simulink model "FeedBack_Linearization"  (R2021b)
(part 3 of 9)

M = ft_5({q1,q2,t10,t1020,t1033,t1034,t1039,t1060,t1066,t1079,t1080,t1090,t1094,t1095,t1097,t1105,t1107,t1116,t1117,t1119,t112,t1120,t1124,t1125,t1131,t1132,t1136,t1140,t1146,t1149,t1151,t1155,t1159,t1168,t1179,t1182,t1183,t1189,t119,t1194,t1197,t1198,t120,t1203,t1204,t121,t1213,t122,t1222,t1229,t1232,t1250,t1255,t1269,t1272,t1282,t1284,t1287,t129,t1292,t1293,t13,t130,t1300,t1307,t1312,t132,t1324,t1327,t1333,t1337,t1338,t1340,t1341,t1342,t1348,t1359,t136,t1364,t1365,t1366,t1368,t1375,t1383,t1394,t1396,t1398,t14,t1403,t1404,t1410,t1414,t1417,t1419,t1425,t1426,t143,t1432,t1446,t1465,t1475,t1486,t1495,t1496,t1498,t1499,t15,t1500,t1501,t1502,t1504,t1505,t1506,t1507,t1510,t1511,t1512,t1513,t1518,t1519,t1522,t1523,t1526,t1529,t153,t1530,t1534,t1535,t1536,t1537,t1542,t1546,t1548,t155,t1550,t1551,t1552,t1555,t1556,t156,t1560,t1561,t1565,t1568,t1569,t1575,t1584,t1589,t1593,t1595,t1598,t16,t1600,t1601,t1603,t1604,t1605,t1606,t1607,t1609,t1610,t1612,t1614,t1615,t1616,t1618,t1620,t1621,t1625,t1626,t1627,t1629,t1631,t1632,t1633,t1637,t164,t1645,t1648,t165,t1653,t1658,t1659,t1662,t1665,t1669,t167,t1671,t1678,t1682,t1685,t1686,t1687,t1689,t1690,t1691,t1695,t1696,t1697,t1699,t17,t170,t1700,t1701,t1702,t1703,t1704,t1707,t1708,t1709,t1710,t1711,t1713,t1715,t1719,t172,t1725,t1726,t1729,t173,t1730,t1731,t1736,t1738,t1741,t1743,t1744,t1749,t1750,t1752,t1753,t1754,t1757,t1758,t1760,t1761,t1762,t1763,t1766,t1767,t1768,t1769,t1771,t1772,t1773,t1776,t1777,t1780,t1782,t1783,t1784,t1785,t1786,t1789,t1790,t1794,t1795,t1797,t1798,t18,t180,t1802,t1803,t1804,t1805,t1806,t1807,t1808,t1809,t1810,t1811,t1812,t1813,t1814,t1815,t1816,t1817,t1818,t1819,t1820,t1821,t1822,t1823,t1824,t1825,t1826,t1827,t1828,t1829,t1831,t1832,t1833,t1835,t1836,t1837,t1839,t1840,t1843,t1844,t1845,t1846,t1847,t1848,t1851,t1852,t1853,t1854,t1855,t1856,t1857,t1858,t1862,t1863,t1867,t1868,t1869,t1870,t1871,t1873,t1874,t1875,t1876,t1877,t1878,t1879,t1883,t1884,t1885,t1888,t1889,t1890,t1892,t1893,t1894,t1895,t1896,t1897,t1900,t1901,t1902,t1903,t1904,t1905,t1906,t1907,t191,t1912,t1913,t1914,t1915,t1916,t1917,t1918,t1919,t1920,t1921,t1922,t1923,t1924,t1925,t1926,t1927,t1929,t1930,t1931,t1932,t1933,t1935,t1937,t1939,t1940,t1941,t1942,t1943,t1944,t1945,t1946,t1947,t1948,t1949,t1950,t1951,t1952,t1953,t1954,t1955,t1956,t1957,t1958,t1959,t1960,t1961,t1962,t1963,t1964,t1965,t1966,t1967,t1969,t1970,t1972,t1973,t1974,t1975,t1976,t1977,t1980,t1981,t1983,t1984,t1985,t1986,t1987,t1990,t1991,t1992,t1993,t1996,t1997,t1998,t1999,t2000,t2001,t2002,t2003,t2004,t2005,t2006,t2007,t2008,t2009,t2011,t2013,t2016,t2017,t2018,t2019,t2021,t2024,t2025,t2027,t2029,t203,t2031,t2032,t2033,t2035,t2036,t2039,t2041,t2043,t2045,t2047,t2048,t2049,t205,t2051,t2054,t2055,t2056,t2057,t2059,t2060,t2062,t2063,t2064,t2065,t2066,t2067,t2068,t2070,t2072,t2073,t2075,t2077,t2079,t2080,t2081,t2082,t2083,t2084,t2088,t2089,t2090,t2091,t2093,t2094,t2095,t2096,t2098,t210,t2101,t2102,t2104,t2106,t2107,t2109,t2111,t2112,t2113,t2114,t2115,t2117,t2118,t2120,t2121,t2122,t2124,t2126,t2128,t2129,t2131,t2132,t2133,t2134,t2135,t2136,t2137,t2139,t2141,t2142,t2145,t2146,t2148,t2149,t2150,t2151,t2152,t2153,t2154,t2156,t2158,t2161,t2162,t2164,t2166,t2168,t2169,t2170,t2172,t2174,t2175,t2176,t2178,t2179,t2182,t2183,t2184,t2187,t2188,t2189,t2190,t2191,t2193,t2194,t2195,t2197,t2201,t2202,t2203,t2204,t2205,t2206,t2208,t2210,t2211,t2212,t2214,t2215,t2216,t2218,t2221,t2222,t2223,t2225,t2226,t2228,t2229,t223,t2231,t2232,t2234,t2235,t2236,t2237,t2239,t2241,t2242,t2244,t2246,t2248,t2249,t225,t2253,t2254,t2255,t2256,t2258,t2259,t2260,t2261,t2262,t2263,t2264,t2266,t2267,t2268,t2269,t227,t2271,t2272,t2273,t2274,t2276,t2278,t228,t2280,t2284,t2287,t2288,t2289,t2295,t2296,t2300,t2301,t2305,t2306,t2309,t231,t2310,t2311,t2313,t2315,t2316,t2318,t2320,t2323,t2324,t2328,t2329,t2331,t2332,t2334,t2335,t2337,t2339,t2340,t2341,t2343,t2344,t2345,t2347,t2348,t2351,t2355,t2356,t2358,t236,t2363,t2364,t2366,t2370,t2371,t2376,t2377,t2378,t2379,t2380,t2383,t2394,t2397,t2401,t2403,t2406,t2409,t2410,t2411,t2413,t2416,t2418,t2419,t2421,t2425,t2427,t2430,t2431,t2434,t2435,t2436,t2439,t2440,t2441,t2442,t2443,t2444,t2445,t2446,t2447,t2450,t2451,t2454,t2456,t2459,t246,t2461,t2462,t2466,t2471,t2472,t2475,t2476,t2478,t2479,t2480,t2492,t2495,t2496,t2497,t2501,t2504,t2505,t2506,t2510,t2511,t2512,t2515,t252,t2522,t2523,t2524,t2527,t2530,t2531,t2536,t2537,t2538,t2542,t2546,t2549,t2550,t2551,t2552,t2554,t2555,t2558,t2559,t2563,t2565,t2566,t257,t2571,t2573,t2575,t273,t277,t300,t308,t31,t311,t312,t313,t314,t315,t32,t328,t33,t333,t342,t346,t36,t395,t396,t397,t451,t452,t455,t470,t485,t5,t500,t51,t515,t53,t533,t544,t55,t565,t57,t580,t6,t614,t639,t648,t654,t655,t66,t671,t673,t675,t679,t68,t7,t703,t710,t711,t717,t725,t726,t727,t748,t75,t765,t769,t770,t773,t788,t795,t8,t822,t826,t836,t854,t856,t865,t87,t873,t888,t889,t890,t896,t9,t902,t909,t910,t914,t929,t930,t933,t938,t942,t944,t969,t977,t979,t98,t980});
end
function M = ft_5(ct)
q1 = ct{1};
q2 = ct{2};
t10 = ct{3};
t1020 = ct{4};
t1033 = ct{5};
t1034 = ct{6};
t1039 = ct{7};
t1060 = ct{8};
t1066 = ct{9};
t1079 = ct{10};
t1080 = ct{11};
t1090 = ct{12};
t1094 = ct{13};
t1095 = ct{14};
t1097 = ct{15};
t1105 = ct{16};
t1107 = ct{17};
t1116 = ct{18};
t1117 = ct{19};
t1119 = ct{20};
t112 = ct{21};
t1120 = ct{22};
t1124 = ct{23};
t1125 = ct{24};
t1131 = ct{25};
t1132 = ct{26};
t1136 = ct{27};
t1140 = ct{28};
t1146 = ct{29};
t1149 = ct{30};
t1151 = ct{31};
t1155 = ct{32};
t1159 = ct{33};
t1168 = ct{34};
t1179 = ct{35};
t1182 = ct{36};
t1183 = ct{37};
t1189 = ct{38};
t119 = ct{39};
t1194 = ct{40};
t1197 = ct{41};
t1198 = ct{42};
t120 = ct{43};
t1203 = ct{44};
t1204 = ct{45};
t121 = ct{46};
t1213 = ct{47};
t122 = ct{48};
t1222 = ct{49};
t1229 = ct{50};
t1232 = ct{51};
t1250 = ct{52};
t1255 = ct{53};
t1269 = ct{54};
t1272 = ct{55};
t1282 = ct{56};
t1284 = ct{57};
t1287 = ct{58};
t129 = ct{59};
t1292 = ct{60};
t1293 = ct{61};
t13 = ct{62};
t130 = ct{63};
t1300 = ct{64};
t1307 = ct{65};
t1312 = ct{66};
t132 = ct{67};
t1324 = ct{68};
t1327 = ct{69};
t1333 = ct{70};
t1337 = ct{71};
t1338 = ct{72};
t1340 = ct{73};
t1341 = ct{74};
t1342 = ct{75};
t1348 = ct{76};
t1359 = ct{77};
t136 = ct{78};
t1364 = ct{79};
t1365 = ct{80};
t1366 = ct{81};
t1368 = ct{82};
t1375 = ct{83};
t1383 = ct{84};
t1394 = ct{85};
t1396 = ct{86};
t1398 = ct{87};
t14 = ct{88};
t1403 = ct{89};
t1404 = ct{90};
t1410 = ct{91};
t1414 = ct{92};
t1417 = ct{93};
t1419 = ct{94};
t1425 = ct{95};
t1426 = ct{96};
t143 = ct{97};
t1432 = ct{98};
t1446 = ct{99};
t1465 = ct{100};
t1475 = ct{101};
t1486 = ct{102};
t1495 = ct{103};
t1496 = ct{104};
t1498 = ct{105};
t1499 = ct{106};
t15 = ct{107};
t1500 = ct{108};
t1501 = ct{109};
t1502 = ct{110};
t1504 = ct{111};
t1505 = ct{112};
t1506 = ct{113};
t1507 = ct{114};
t1510 = ct{115};
t1511 = ct{116};
t1512 = ct{117};
t1513 = ct{118};
t1518 = ct{119};
t1519 = ct{120};
t1522 = ct{121};
t1523 = ct{122};
t1526 = ct{123};
t1529 = ct{124};
t153 = ct{125};
t1530 = ct{126};
t1534 = ct{127};
t1535 = ct{128};
t1536 = ct{129};
t1537 = ct{130};
t1542 = ct{131};
t1546 = ct{132};
t1548 = ct{133};
t155 = ct{134};
t1550 = ct{135};
t1551 = ct{136};
t1552 = ct{137};
t1555 = ct{138};
t1556 = ct{139};
t156 = ct{140};
t1560 = ct{141};
t1561 = ct{142};
t1565 = ct{143};
t1568 = ct{144};
t1569 = ct{145};
t1575 = ct{146};
t1584 = ct{147};
t1589 = ct{148};
t1593 = ct{149};
t1595 = ct{150};
t1598 = ct{151};
t16 = ct{152};
t1600 = ct{153};
t1601 = ct{154};
t1603 = ct{155};
t1604 = ct{156};
t1605 = ct{157};
t1606 = ct{158};
t1607 = ct{159};
t1609 = ct{160};
t1610 = ct{161};
t1612 = ct{162};
t1614 = ct{163};
t1615 = ct{164};
t1616 = ct{165};
t1618 = ct{166};
t1620 = ct{167};
t1621 = ct{168};
t1625 = ct{169};
t1626 = ct{170};
t1627 = ct{171};
t1629 = ct{172};
t1631 = ct{173};
t1632 = ct{174};
t1633 = ct{175};
t1637 = ct{176};
t164 = ct{177};
t1645 = ct{178};
t1648 = ct{179};
t165 = ct{180};
t1653 = ct{181};
t1658 = ct{182};
t1659 = ct{183};
t1662 = ct{184};
t1665 = ct{185};
t1669 = ct{186};
t167 = ct{187};
t1671 = ct{188};
t1678 = ct{189};
t1682 = ct{190};
t1685 = ct{191};
t1686 = ct{192};
t1687 = ct{193};
t1689 = ct{194};
t1690 = ct{195};
t1691 = ct{196};
t1695 = ct{197};
t1696 = ct{198};
t1697 = ct{199};
t1699 = ct{200};
t17 = ct{201};
t170 = ct{202};
t1700 = ct{203};
t1701 = ct{204};
t1702 = ct{205};
t1703 = ct{206};
t1704 = ct{207};
t1707 = ct{208};
t1708 = ct{209};
t1709 = ct{210};
t1710 = ct{211};
t1711 = ct{212};
t1713 = ct{213};
t1715 = ct{214};
t1719 = ct{215};
t172 = ct{216};
t1725 = ct{217};
t1726 = ct{218};
t1729 = ct{219};
t173 = ct{220};
t1730 = ct{221};
t1731 = ct{222};
t1736 = ct{223};
t1738 = ct{224};
t1741 = ct{225};
t1743 = ct{226};
t1744 = ct{227};
t1749 = ct{228};
t1750 = ct{229};
t1752 = ct{230};
t1753 = ct{231};
t1754 = ct{232};
t1757 = ct{233};
t1758 = ct{234};
t1760 = ct{235};
t1761 = ct{236};
t1762 = ct{237};
t1763 = ct{238};
t1766 = ct{239};
t1767 = ct{240};
t1768 = ct{241};
t1769 = ct{242};
t1771 = ct{243};
t1772 = ct{244};
t1773 = ct{245};
t1776 = ct{246};
t1777 = ct{247};
t1780 = ct{248};
t1782 = ct{249};
t1783 = ct{250};
t1784 = ct{251};
t1785 = ct{252};
t1786 = ct{253};
t1789 = ct{254};
t1790 = ct{255};
t1794 = ct{256};
t1795 = ct{257};
t1797 = ct{258};
t1798 = ct{259};
t18 = ct{260};
t180 = ct{261};
t1802 = ct{262};
t1803 = ct{263};
t1804 = ct{264};
t1805 = ct{265};
t1806 = ct{266};
t1807 = ct{267};
t1808 = ct{268};
t1809 = ct{269};
t1810 = ct{270};
t1811 = ct{271};
t1812 = ct{272};
t1813 = ct{273};
t1814 = ct{274};
t1815 = ct{275};
t1816 = ct{276};
t1817 = ct{277};
t1818 = ct{278};
t1819 = ct{279};
t1820 = ct{280};
t1821 = ct{281};
t1822 = ct{282};
t1823 = ct{283};
t1824 = ct{284};
t1825 = ct{285};
t1826 = ct{286};
t1827 = ct{287};
t1828 = ct{288};
t1829 = ct{289};
t1831 = ct{290};
t1832 = ct{291};
t1833 = ct{292};
t1835 = ct{293};
t1836 = ct{294};
t1837 = ct{295};
t1839 = ct{296};
t1840 = ct{297};
t1843 = ct{298};
t1844 = ct{299};
t1845 = ct{300};
t1846 = ct{301};
t1847 = ct{302};
t1848 = ct{303};
t1851 = ct{304};
t1852 = ct{305};
t1853 = ct{306};
t1854 = ct{307};
t1855 = ct{308};
t1856 = ct{309};
t1857 = ct{310};
t1858 = ct{311};
t1862 = ct{312};
t1863 = ct{313};
t1867 = ct{314};
t1868 = ct{315};
t1869 = ct{316};
t1870 = ct{317};
t1871 = ct{318};
t1873 = ct{319};
t1874 = ct{320};
t1875 = ct{321};
t1876 = ct{322};
t1877 = ct{323};
t1878 = ct{324};
t1879 = ct{325};
t1883 = ct{326};
t1884 = ct{327};
t1885 = ct{328};
t1888 = ct{329};
t1889 = ct{330};
t1890 = ct{331};
t1892 = ct{332};
t1893 = ct{333};
t1894 = ct{334};
t1895 = ct{335};
t1896 = ct{336};
t1897 = ct{337};
t1900 = ct{338};
t1901 = ct{339};
t1902 = ct{340};
t1903 = ct{341};
t1904 = ct{342};
t1905 = ct{343};
t1906 = ct{344};
t1907 = ct{345};
t191 = ct{346};
t1912 = ct{347};
t1913 = ct{348};
t1914 = ct{349};
t1915 = ct{350};
t1916 = ct{351};
t1917 = ct{352};
t1918 = ct{353};
t1919 = ct{354};
t1920 = ct{355};
t1921 = ct{356};
t1922 = ct{357};
t1923 = ct{358};
t1924 = ct{359};
t1925 = ct{360};
t1926 = ct{361};
t1927 = ct{362};
t1929 = ct{363};
t1930 = ct{364};
t1931 = ct{365};
t1932 = ct{366};
t1933 = ct{367};
t1935 = ct{368};
t1937 = ct{369};
t1939 = ct{370};
t1940 = ct{371};
t1941 = ct{372};
t1942 = ct{373};
t1943 = ct{374};
t1944 = ct{375};
t1945 = ct{376};
t1946 = ct{377};
t1947 = ct{378};
t1948 = ct{379};
t1949 = ct{380};
t1950 = ct{381};
t1951 = ct{382};
t1952 = ct{383};
t1953 = ct{384};
t1954 = ct{385};
t1955 = ct{386};
t1956 = ct{387};
t1957 = ct{388};
t1958 = ct{389};
t1959 = ct{390};
t1960 = ct{391};
t1961 = ct{392};
t1962 = ct{393};
t1963 = ct{394};
t1964 = ct{395};
t1965 = ct{396};
t1966 = ct{397};
t1967 = ct{398};
t1969 = ct{399};
t1970 = ct{400};
t1972 = ct{401};
t1973 = ct{402};
t1974 = ct{403};
t1975 = ct{404};
t1976 = ct{405};
t1977 = ct{406};
t1980 = ct{407};
t1981 = ct{408};
t1983 = ct{409};
t1984 = ct{410};
t1985 = ct{411};
t1986 = ct{412};
t1987 = ct{413};
t1990 = ct{414};
t1991 = ct{415};
t1992 = ct{416};
t1993 = ct{417};
t1996 = ct{418};
t1997 = ct{419};
t1998 = ct{420};
t1999 = ct{421};
t2000 = ct{422};
t2001 = ct{423};
t2002 = ct{424};
t2003 = ct{425};
t2004 = ct{426};
t2005 = ct{427};
t2006 = ct{428};
t2007 = ct{429};
t2008 = ct{430};
t2009 = ct{431};
t2011 = ct{432};
t2013 = ct{433};
t2016 = ct{434};
t2017 = ct{435};
t2018 = ct{436};
t2019 = ct{437};
t2021 = ct{438};
t2024 = ct{439};
t2025 = ct{440};
t2027 = ct{441};
t2029 = ct{442};
t203 = ct{443};
t2031 = ct{444};
t2032 = ct{445};
t2033 = ct{446};
t2035 = ct{447};
t2036 = ct{448};
t2039 = ct{449};
t2041 = ct{450};
t2043 = ct{451};
t2045 = ct{452};
t2047 = ct{453};
t2048 = ct{454};
t2049 = ct{455};
t205 = ct{456};
t2051 = ct{457};
t2054 = ct{458};
t2055 = ct{459};
t2056 = ct{460};
t2057 = ct{461};
t2059 = ct{462};
t2060 = ct{463};
t2062 = ct{464};
t2063 = ct{465};
t2064 = ct{466};
t2065 = ct{467};
t2066 = ct{468};
t2067 = ct{469};
t2068 = ct{470};
t2070 = ct{471};
t2072 = ct{472};
t2073 = ct{473};
t2075 = ct{474};
t2077 = ct{475};
t2079 = ct{476};
t2080 = ct{477};
t2081 = ct{478};
t2082 = ct{479};
t2083 = ct{480};
t2084 = ct{481};
t2088 = ct{482};
t2089 = ct{483};
t2090 = ct{484};
t2091 = ct{485};
t2093 = ct{486};
t2094 = ct{487};
t2095 = ct{488};
t2096 = ct{489};
t2098 = ct{490};
t210 = ct{491};
t2101 = ct{492};
t2102 = ct{493};
t2104 = ct{494};
t2106 = ct{495};
t2107 = ct{496};
t2109 = ct{497};
t2111 = ct{498};
t2112 = ct{499};
t2113 = ct{500};
t2114 = ct{501};
t2115 = ct{502};
t2117 = ct{503};
t2118 = ct{504};
t2120 = ct{505};
t2121 = ct{506};
t2122 = ct{507};
t2124 = ct{508};
t2126 = ct{509};
t2128 = ct{510};
t2129 = ct{511};
t2131 = ct{512};
t2132 = ct{513};
t2133 = ct{514};
t2134 = ct{515};
t2135 = ct{516};
t2136 = ct{517};
t2137 = ct{518};
t2139 = ct{519};
t2141 = ct{520};
t2142 = ct{521};
t2145 = ct{522};
t2146 = ct{523};
t2148 = ct{524};
t2149 = ct{525};
t2150 = ct{526};
t2151 = ct{527};
t2152 = ct{528};
t2153 = ct{529};
t2154 = ct{530};
t2156 = ct{531};
t2158 = ct{532};
t2161 = ct{533};
t2162 = ct{534};
t2164 = ct{535};
t2166 = ct{536};
t2168 = ct{537};
t2169 = ct{538};
t2170 = ct{539};
t2172 = ct{540};
t2174 = ct{541};
t2175 = ct{542};
t2176 = ct{543};
t2178 = ct{544};
t2179 = ct{545};
t2182 = ct{546};
t2183 = ct{547};
t2184 = ct{548};
t2187 = ct{549};
t2188 = ct{550};
t2189 = ct{551};
t2190 = ct{552};
t2191 = ct{553};
t2193 = ct{554};
t2194 = ct{555};
t2195 = ct{556};
t2197 = ct{557};
t2201 = ct{558};
t2202 = ct{559};
t2203 = ct{560};
t2204 = ct{561};
t2205 = ct{562};
t2206 = ct{563};
t2208 = ct{564};
t2210 = ct{565};
t2211 = ct{566};
t2212 = ct{567};
t2214 = ct{568};
t2215 = ct{569};
t2216 = ct{570};
t2218 = ct{571};
t2221 = ct{572};
t2222 = ct{573};
t2223 = ct{574};
t2225 = ct{575};
t2226 = ct{576};
t2228 = ct{577};
t2229 = ct{578};
t223 = ct{579};
t2231 = ct{580};
t2232 = ct{581};
t2234 = ct{582};
t2235 = ct{583};
t2236 = ct{584};
t2237 = ct{585};
t2239 = ct{586};
t2241 = ct{587};
t2242 = ct{588};
t2244 = ct{589};
t2246 = ct{590};
t2248 = ct{591};
t2249 = ct{592};
t225 = ct{593};
t2253 = ct{594};
t2254 = ct{595};
t2255 = ct{596};
t2256 = ct{597};
t2258 = ct{598};
t2259 = ct{599};
t2260 = ct{600};
t2261 = ct{601};
t2262 = ct{602};
t2263 = ct{603};
t2264 = ct{604};
t2266 = ct{605};
t2267 = ct{606};
t2268 = ct{607};
t2269 = ct{608};
t227 = ct{609};
t2271 = ct{610};
t2272 = ct{611};
t2273 = ct{612};
t2274 = ct{613};
t2276 = ct{614};
t2278 = ct{615};
t228 = ct{616};
t2280 = ct{617};
t2284 = ct{618};
t2287 = ct{619};
t2288 = ct{620};
t2289 = ct{621};
t2295 = ct{622};
t2296 = ct{623};
t2300 = ct{624};
t2301 = ct{625};
t2305 = ct{626};
t2306 = ct{627};
t2309 = ct{628};
t231 = ct{629};
t2310 = ct{630};
t2311 = ct{631};
t2313 = ct{632};
t2315 = ct{633};
t2316 = ct{634};
t2318 = ct{635};
t2320 = ct{636};
t2323 = ct{637};
t2324 = ct{638};
t2328 = ct{639};
t2329 = ct{640};
t2331 = ct{641};
t2332 = ct{642};
t2334 = ct{643};
t2335 = ct{644};
t2337 = ct{645};
t2339 = ct{646};
t2340 = ct{647};
t2341 = ct{648};
t2343 = ct{649};
t2344 = ct{650};
t2345 = ct{651};
t2347 = ct{652};
t2348 = ct{653};
t2351 = ct{654};
t2355 = ct{655};
t2356 = ct{656};
t2358 = ct{657};
t236 = ct{658};
t2363 = ct{659};
t2364 = ct{660};
t2366 = ct{661};
t2370 = ct{662};
t2371 = ct{663};
t2376 = ct{664};
t2377 = ct{665};
t2378 = ct{666};
t2379 = ct{667};
t2380 = ct{668};
t2383 = ct{669};
t2394 = ct{670};
t2397 = ct{671};
t2401 = ct{672};
t2403 = ct{673};
t2406 = ct{674};
t2409 = ct{675};
t2410 = ct{676};
t2411 = ct{677};
t2413 = ct{678};
t2416 = ct{679};
t2418 = ct{680};
t2419 = ct{681};
t2421 = ct{682};
t2425 = ct{683};
t2427 = ct{684};
t2430 = ct{685};
t2431 = ct{686};
t2434 = ct{687};
t2435 = ct{688};
t2436 = ct{689};
t2439 = ct{690};
t2440 = ct{691};
t2441 = ct{692};
t2442 = ct{693};
t2443 = ct{694};
t2444 = ct{695};
t2445 = ct{696};
t2446 = ct{697};
t2447 = ct{698};
t2450 = ct{699};
t2451 = ct{700};
t2454 = ct{701};
t2456 = ct{702};
t2459 = ct{703};
t246 = ct{704};
t2461 = ct{705};
t2462 = ct{706};
t2466 = ct{707};
t2471 = ct{708};
t2472 = ct{709};
t2475 = ct{710};
t2476 = ct{711};
t2478 = ct{712};
t2479 = ct{713};
t2480 = ct{714};
t2492 = ct{715};
t2495 = ct{716};
t2496 = ct{717};
t2497 = ct{718};
t2501 = ct{719};
t2504 = ct{720};
t2505 = ct{721};
t2506 = ct{722};
t2510 = ct{723};
t2511 = ct{724};
t2512 = ct{725};
t2515 = ct{726};
t252 = ct{727};
t2522 = ct{728};
t2523 = ct{729};
t2524 = ct{730};
t2527 = ct{731};
t2530 = ct{732};
t2531 = ct{733};
t2536 = ct{734};
t2537 = ct{735};
t2538 = ct{736};
t2542 = ct{737};
t2546 = ct{738};
t2549 = ct{739};
t2550 = ct{740};
t2551 = ct{741};
t2552 = ct{742};
t2554 = ct{743};
t2555 = ct{744};
t2558 = ct{745};
t2559 = ct{746};
t2563 = ct{747};
t2565 = ct{748};
t2566 = ct{749};
t257 = ct{750};
t2571 = ct{751};
t2573 = ct{752};
t2575 = ct{753};
t273 = ct{754};
t277 = ct{755};
t300 = ct{756};
t308 = ct{757};
t31 = ct{758};
t311 = ct{759};
t312 = ct{760};
t313 = ct{761};
t314 = ct{762};
t315 = ct{763};
t32 = ct{764};
t328 = ct{765};
t33 = ct{766};
t333 = ct{767};
t342 = ct{768};
t346 = ct{769};
t36 = ct{770};
t395 = ct{771};
t396 = ct{772};
t397 = ct{773};
t451 = ct{774};
t452 = ct{775};
t455 = ct{776};
t470 = ct{777};
t485 = ct{778};
t5 = ct{779};
t500 = ct{780};
t51 = ct{781};
t515 = ct{782};
t53 = ct{783};
t533 = ct{784};
t544 = ct{785};
t55 = ct{786};
t565 = ct{787};
t57 = ct{788};
t580 = ct{789};
t6 = ct{790};
t614 = ct{791};
t639 = ct{792};
t648 = ct{793};
t654 = ct{794};
t655 = ct{795};
t66 = ct{796};
t671 = ct{797};
t673 = ct{798};
t675 = ct{799};
t679 = ct{800};
t68 = ct{801};
t7 = ct{802};
t703 = ct{803};
t710 = ct{804};
t711 = ct{805};
t717 = ct{806};
t725 = ct{807};
t726 = ct{808};
t727 = ct{809};
t748 = ct{810};
t75 = ct{811};
t765 = ct{812};
t769 = ct{813};
t770 = ct{814};
t773 = ct{815};
t788 = ct{816};
t795 = ct{817};
t8 = ct{818};
t822 = ct{819};
t826 = ct{820};
t836 = ct{821};
t854 = ct{822};
t856 = ct{823};
t865 = ct{824};
t87 = ct{825};
t873 = ct{826};
t888 = ct{827};
t889 = ct{828};
t890 = ct{829};
t896 = ct{830};
t9 = ct{831};
t902 = ct{832};
t909 = ct{833};
t910 = ct{834};
t914 = ct{835};
t929 = ct{836};
t930 = ct{837};
t933 = ct{838};
t938 = ct{839};
t942 = ct{840};
t944 = ct{841};
t969 = ct{842};
t977 = ct{843};
t979 = ct{844};
t98 = ct{845};
t980 = ct{846};
t2577 = t2478.*(-t826+t856.*(t129+t13.*(t51-t155))+t836.*(t156-t236)).*(-1.0./2.0);
et77 = t1394.*4.000000000000028e-5+t1518+t1530+t1593+t1709+t565.*(t129+t13.*(t51-t155)).*5.0e-5;
et78 = t225.*(t136-t246).*2.81e-3+t452.*(t57-t165).*5.0e-5;
et79 = t856.*(t66-t210).*2.81e-3;
t2580 = t1967.*(et77+et78+et79).*(-1.0./2.0);
et80 = t1394.*4.000000000000028e-5+t1518+t1530+t1593+t1709+t565.*(t129+t13.*(t51-t155)).*5.0e-5;
et81 = t225.*(t136-t246).*2.81e-3+t452.*(t57-t165).*5.0e-5;
et82 = t856.*(t66-t210).*2.81e-3;
t2581 = (t1967.*(et80+et81+et82))./2.0;
et83 = t1537+t1575+t1704-t1710+t396.*(t167+t7.*(t55-t130)).*3.0e-5+t565.*(t129+t13.*(t51-t155)).*5.000000000000004e-4;
et84 = t225.*(t136-t246).*5.0e-5+t452.*(t57-t165).*5.000000000000004e-4;
et85 = t856.*(t66-t210).*5.0e-5;
t2582 = ((et83+et84+et85).*(-t826+t856.*(t129+t13.*(t51-t155))+t836.*(t156-t236)))./2.0;
et86 = t710.*4.000000000000028e-5-t1375+t1486+t1535+t1542+t671.*(t129+t13.*(t51-t155)).*3.0e-5;
et87 = t655.*(t485+t7.*(t53-t132)).*2.32e-3+t888.*(t273+t14.*(t51-t155)).*2.32e-3;
et88 = t614.*(t156-t236).*3.0e-5;
t2584 = t1986.*(et86+et87+et88).*(-1.0./2.0);
et89 = t710.*4.000000000000028e-5-t1375+t1486+t1535+t1542+t671.*(t129+t13.*(t51-t155)).*3.0e-5;
et90 = t655.*(t485+t7.*(t53-t132)).*2.32e-3+t888.*(t273+t14.*(t51-t155)).*2.32e-3;
et91 = t614.*(t156-t236).*3.0e-5;
t2586 = (t1986.*(et89+et90+et91))./2.0;
et92 = t710.*4.000000000000028e-5-t1375+t1486+t1535+t1542+t671.*(t129+t13.*(t51-t155)).*3.0e-5;
et93 = t655.*(t485+t7.*(t53-t132)).*2.32e-3+t888.*(t273+t14.*(t51-t155)).*2.32e-3;
et94 = t614.*(t156-t236).*3.0e-5;
t2590 = t1990.*(et92+et93+et94).*(-1.0./2.0);
t1712 = -t1708;
t1714 = -t1711;
t1722 = -t1719;
t1733 = -t1726;
t1740 = -t1730;
t1746 = -t1741;
t1859 = -t1855;
t1860 = -t1856;
t1861 = -t1857;
t1864 = -t1858;
t1865 = -t1862;
t1866 = -t1863;
t1880 = -t1877;
t1881 = -t1878;
t1882 = -t1879;
t1898 = -t1893;
t1899 = -t1896;
t1908 = -t1901;
t1909 = -t1903;
t1910 = -t1904;
t1911 = -t1906;
t1934 = -t1932;
t1936 = -t1933;
t1938 = -t1937;
t1978 = -t1974;
t1979 = -t1976;
t1982 = -t1980;
t2012 = t1750+t1753;
t2014 = t1761+t1762;
t2050 = t1348+t1614+t1631;
t2069 = t1871+t1876;
t2125 = t1519+t1786+t1790;
t2180 = -t2179;
t2250 = t2006.*t2016.*3.5432e-1;
t2265 = t2006.*t2027.*3.5432e-1;
t2281 = t2003.*t2065.*3.5432e-1;
t2283 = t2006.*t2067.*3.5432e-1;
t2286 = -t2284;
t2290 = t2009.*t2065.*3.5432e-1;
t2291 = t2006.*t2072.*3.5432e-1;
t2292 = t2006.*(t203-t679+t725.*2.324e-2+t865+t873+t1146+t14.*(t143-t164).*1.9738e-1).*(-3.5432e-1);
t2294 = t2006.*(t203-t679+t725.*2.324e-2+t865+t873+t1146+t14.*(t143-t164).*1.9738e-1).*3.5432e-1;
t2297 = -t2296;
t2298 = t2016.*t2067.*3.5432e-1;
t2302 = -t2300;
t2304 = -t2301;
t2314 = t2019.*t2065.*3.5432e-1;
t2321 = t2027.*t2067.*3.5432e-1;
t2325 = -t2324;
t2346 = t2006.*t2126.*3.5432e-1;
t2349 = t2003.*t2136.*3.5432e-1;
t2352 = t2057.*t2065.*3.5432e-1;
t2359 = t2016.*t2126.*3.5432e-1;
t2360 = t2009.*t2136.*3.5432e-1;
t2361 = t2067.*t2072.*3.5432e-1;
t2362 = t2067.*(t203-t679+t725.*2.324e-2+t865+t873+t1146+t14.*(t143-t164).*1.9738e-1).*(-3.5432e-1);
t2365 = t2065.*t2082.*3.5432e-1;
t2372 = (t1398.*t2287)./2.0;
t2373 = t2027.*t2126.*3.5432e-1;
t2374 = t2019.*t2136.*3.5432e-1;
t2382 = t2067.*t2126.*3.5432e-1;
t2385 = t2057.*t2136.*3.5432e-1;
t2387 = t2072.*t2126.*3.5432e-1;
t2389 = t2126.*(t203-t679+t725.*2.324e-2+t865+t873+t1146+t14.*(t143-t164).*1.9738e-1).*(-3.5432e-1);
t2390 = t2126.*(t203-t679+t725.*2.324e-2+t865+t873+t1146+t14.*(t143-t164).*1.9738e-1).*3.5432e-1;
t2391 = t2065.*t2136.*3.5432e-1;
t2392 = t2082.*t2136.*3.5432e-1;
t2395 = (t1826.*t2280)./2.0;
t2398 = t2287.*(t1333+t888.*(t156-t236)).*(-1.0./2.0);
t2399 = (t2287.*(t1333+t888.*(t156-t236)))./2.0;
t2404 = (t1884.*t2280)./2.0;
t2408 = t2287.*(t639+t648.*(t129+t13.*(t51-t155))+t673.*(t156-t236)).*(-1.0./2.0);
t2414 = t2287.*(-t726+t671.*(t129+t13.*(t51-t155))+t614.*(t156-t236)).*(-1.0./2.0);
t2415 = t2287.*(t1107+t565.*(t129+t13.*(t51-t155))+t452.*(t57-t165)).*(-1.0./2.0);
t2420 = t2280.*(t1189+t225.*(t136-t246)+t856.*(t66-t210)).*(-1.0./2.0);
t2422 = (t1929.*t2280)./2.0;
t2423 = (t2280.*(t1189+t225.*(t136-t246)+t856.*(t66-t210)))./2.0;
t2429 = (t1967.*t2280)./2.0;
t2432 = (t1966.*t2288)./2.0;
t2437 = (t1973.*t2288)./2.0;
t2448 = (t1986.*t2288)./2.0;
t2452 = t2288.*(t890+t655.*(t485+t7.*(t53-t132))+t888.*(t273+t14.*(t51-t155))).*(-1.0./2.0);
t2453 = (t1990.*t2288)./2.0;
t2460 = (t1398.*t2413)./2.0;
t2464 = (t1738.*t2406)./2.0;
t2467 = t2413.*(t639+t648.*(t129+t13.*(t51-t155))+t673.*(t156-t236)).*(-1.0./2.0);
t2468 = t2413.*(-t726+t671.*(t129+t13.*(t51-t155))+t614.*(t156-t236)).*(-1.0./2.0);
t2469 = t2413.*(t1107+t565.*(t129+t13.*(t51-t155))+t452.*(t57-t165)).*(-1.0./2.0);
t2473 = -t2471;
t2482 = t1426+t1446+t1522+t1534+t1536+t1598+t1600+t1700+t1713;
t2483 = t1768.*(t1499+t1711+t1726-t1924+t396.*(t515+t15.*(t57-t165)).*7.950000000000001e-3+t1359.*(t485+t7.*(t53-t132)).*7.950000000000001e-3).*(-1.0./2.0);
t2484 = t2413.*(-t826+t856.*(t129+t13.*(t51-t155))+t836.*(t156-t236)).*(-1.0./2.0);
t2485 = (t2413.*(-t826+t856.*(t129+t13.*(t51-t155))+t836.*(t156-t236)))./2.0;
t2486 = (t1973.*t2406)./2.0;
t2488 = (t1986.*t2406)./2.0;
t2490 = t2406.*(t890+t655.*(t485+t7.*(t53-t132))+t888.*(t273+t14.*(t51-t155))).*(-1.0./2.0);
t2491 = (t1990.*t2406)./2.0;
t2493 = (t1826.*t2462)./2.0;
t2498 = -t2497;
t2499 = (t1884.*t2462)./2.0;
t2507 = t2462.*(t1189+t225.*(t136-t246)+t856.*(t66-t210)).*(-1.0./2.0);
t2508 = (t1929.*t2462)./2.0;
t2513 = (t1738.*t2476)./2.0;
t2516 = -t2515;
t2517 = (t1738.*t2479)./2.0;
t2518 = ((t1752+t1383.*(t485+t7.*(t53-t132))).*(t1495+t1708+t1730-t1921+t396.*(t515+t15.*(t57-t165)).*2.2e-4+t1359.*(t485+t7.*(t53-t132)).*2.2e-4))./2.0;
et95 = (t1743+t1368.*(t485+t7.*(t53-t132))).*(t1499+t1711+t1726-t1924+t396.*(t515+t15.*(t57-t165)).*7.950000000000001e-3+t1359.*(t485+t7.*(t53-t132)).*7.950000000000001e-3);
et96 = 1.0./2.0;
t2520 = et95.*et96;
t2525 = -t2524;
et97 = t1120+t1060.*(t485+t7.*(t53-t132))+t888.*(t257+t15.*(t273+t14.*(t51-t155)));
et98 = (t1499+t1711+t1726-t1924+t396.*(t515+t15.*(t57-t165)).*7.950000000000001e-3+t1359.*(t485+t7.*(t53-t132)).*7.950000000000001e-3)./2.0;
t2528 = et97.*et98;
t2539 = t2032.*(t1499+t1711+t1726-t1924+t396.*(t515+t15.*(t57-t165)).*7.950000000000001e-3+t1359.*(t485+t7.*(t53-t132)).*7.950000000000001e-3).*(-1.0./2.0);
et99 = t1203+t14.*t1383.*(t129+t13.*(t51-t155))+t14.*t1359.*(t156-t236);
et100 = (t1495+t1708+t1730-t1921+t396.*(t515+t15.*(t57-t165)).*2.2e-4+t1359.*(t485+t7.*(t53-t132)).*2.2e-4)./2.0;
t2540 = et99.*et100;
t2541 = -t2538;
et101 = t1179-t1618+t1105.*(t485+t7.*(t53-t132));
et102 = (t1499+t1711+t1726-t1924+t396.*(t515+t15.*(t57-t165)).*7.950000000000001e-3+t1359.*(t485+t7.*(t53-t132)).*7.950000000000001e-3)./2.0;
t2544 = et101.*et102;
t2545 = t2035.*(t1499+t1711+t1726-t1924+t396.*(t515+t15.*(t57-t165)).*7.950000000000001e-3+t1359.*(t485+t7.*(t53-t132)).*7.950000000000001e-3).*(-1.0./2.0);
t2553 = -t2552;
t2556 = t2049.*(t1495+t1708+t1730-t1921+t396.*(t515+t15.*(t57-t165)).*2.2e-4+t1359.*(t485+t7.*(t53-t132)).*2.2e-4).*(-1.0./2.0);
t2557 = (t2049.*(t1495+t1708+t1730-t1921+t396.*(t515+t15.*(t57-t165)).*2.2e-4+t1359.*(t485+t7.*(t53-t132)).*2.2e-4))./2.0;
et103 = (-t1614+t1626+t452.*(t515+t15.*(t57-t165))).*(t1495+t1708+t1730-t1921+t396.*(t515+t15.*(t57-t165)).*2.2e-4+t1359.*(t485+t7.*(t53-t132)).*2.2e-4);
et104 = 1.0./2.0;
t2560 = et103.*et104;
t2561 = t2051.*(t1495+t1708+t1730-t1921+t396.*(t515+t15.*(t57-t165)).*2.2e-4+t1359.*(t485+t7.*(t53-t132)).*2.2e-4).*(-1.0./2.0);
t2562 = (t2051.*(t1495+t1708+t1730-t1921+t396.*(t515+t15.*(t57-t165)).*2.2e-4+t1359.*(t485+t7.*(t53-t132)).*2.2e-4))./2.0;
t2567 = -t2566;
t2568 = (t1966.*t2476)./2.0;
t2576 = (t1966.*t2479)./2.0;
t2579 = (t1973.*t2476)./2.0;
t2583 = -t2582;
t2585 = (t1973.*t2479)./2.0;
t2587 = t2084.*(t1495+t1708+t1730-t1921+t396.*(t515+t15.*(t57-t165)).*2.2e-4+t1359.*(t485+t7.*(t53-t132)).*2.2e-4).*(-1.0./2.0);
t2589 = t2088.*(t1507+t1719+t1741-t1923+t396.*(t515+t15.*(t57-t165)).*2.900000000000001e-4+t1359.*(t485+t7.*(t53-t132)).*2.900000000000001e-4).*(-1.0./2.0);
t2591 = t2476.*(t890+t655.*(t485+t7.*(t53-t132))+t888.*(t273+t14.*(t51-t155))).*(-1.0./2.0);
t2592 = (t2476.*(t890+t655.*(t485+t7.*(t53-t132))+t888.*(t273+t14.*(t51-t155))))./2.0;
t2593 = (t1990.*t2476)./2.0;
t2595 = (t1986.*t2479)./2.0;
t2597 = t2479.*(t890+t655.*(t485+t7.*(t53-t132))+t888.*(t273+t14.*(t51-t155))).*(-1.0./2.0);
t2598 = t2113.*(t1507+t1719+t1741-t1923+t396.*(t515+t15.*(t57-t165)).*2.900000000000001e-4+t1359.*(t485+t7.*(t53-t132)).*2.900000000000001e-4).*(-1.0./2.0);
t2599 = t2120.*(t1507+t1719+t1741-t1923+t396.*(t515+t15.*(t57-t165)).*2.900000000000001e-4+t1359.*(t485+t7.*(t53-t132)).*2.900000000000001e-4).*(-1.0./2.0);
t2600 = t2121.*(t1507+t1719+t1741-t1923+t396.*(t515+t15.*(t57-t165)).*2.900000000000001e-4+t1359.*(t485+t7.*(t53-t132)).*2.900000000000001e-4).*(-1.0./2.0);
t2601 = (t2120.*(t1507+t1719+t1741-t1923+t396.*(t515+t15.*(t57-t165)).*2.900000000000001e-4+t1359.*(t485+t7.*(t53-t132)).*2.900000000000001e-4))./2.0;
t2602 = (t2121.*(t1507+t1719+t1741-t1923+t396.*(t515+t15.*(t57-t165)).*2.900000000000001e-4+t1359.*(t485+t7.*(t53-t132)).*2.900000000000001e-4))./2.0;
et105 = t1780-t1790+t889.*(t8.*(t57-t165)+t15.*(t136-t246));
et106 = (t1507+t1719+t1741-t1923+t396.*(t515+t15.*(t57-t165)).*2.900000000000001e-4+t1359.*(t485+t7.*(t53-t132)).*2.900000000000001e-4)./2.0;
t2603 = et105.*et106;
t2604 = t1282+t1496+t1511+t1686+t1701+t1888+t1895+t1913+t1920;
t2605 = t1287+t1498+t1506+t1702+t1703+t1889+t1907+t1914+t1925;
t2606 = t1307+t1510+t1513+t1685+t1696+t1890+t1892+t1917+t1922;
t2607 = t1768.*(t1901+t1906+t1974-t1975+t1368.*(t485+t7.*(t53-t132)).*7.950000000000001e-3+t1383.*(t485+t7.*(t53-t132)).*2.2e-4).*(-1.0./2.0);
t2608 = (t1768.*(t1901+t1906+t1974-t1975+t1368.*(t485+t7.*(t53-t132)).*7.950000000000001e-3+t1383.*(t485+t7.*(t53-t132)).*2.2e-4))./2.0;
t2609 = t1984.*(t1893+t1904+t1980-t1981+t1368.*(t485+t7.*(t53-t132)).*2.900000000000001e-4+t1383.*(t485+t7.*(t53-t132)).*2.9e-4).*(-1.0./2.0);
t2613 = t1584+t1609+t1758+t1820+t1827+t1836+t1846+t1942+t1957;
t2614 = t1589+t1610+t1767+t1821+t1824+t1837+t1843+t1946+t1963;
t2615 = t1595+t1612+t1763+t1818+t1829+t1840+t1854+t1940+t1955;
t2616 = t1548+t1615+t1725+t1844+t1845+t1868+t1873+t1951+t1956;
t2617 = t1551+t1616+t1744+t1847+t1848+t1869+t1874+t1958+t1962;
t2618 = t1561+t1620+t1729+t1852+t1853+t1870+t1875+t1950+t1959;
et107 = t1120+t1060.*(t485+t7.*(t53-t132))+t888.*(t257+t15.*(t273+t14.*(t51-t155)));
et108 = (t1901+t1906+t1974-t1975+t1368.*(t485+t7.*(t53-t132)).*7.950000000000001e-3+t1383.*(t485+t7.*(t53-t132)).*2.2e-4)./2.0;
t2622 = et107.*et108;
t2624 = t2032.*(t1901+t1906+t1974-t1975+t1368.*(t485+t7.*(t53-t132)).*7.950000000000001e-3+t1383.*(t485+t7.*(t53-t132)).*2.2e-4).*(-1.0./2.0);
t2625 = (t2032.*(t1901+t1906+t1974-t1975+t1368.*(t485+t7.*(t53-t132)).*7.950000000000001e-3+t1383.*(t485+t7.*(t53-t132)).*2.2e-4))./2.0;
et109 = t1203+t14.*t1383.*(t129+t13.*(t51-t155))+t14.*t1359.*(t156-t236);
et110 = (t1896+t1903+t1976-t1977+t1368.*(t485+t7.*(t53-t132)).*2.2e-4+t1383.*(t485+t7.*(t53-t132)).*1.089e-2)./2.0;
t2626 = et109.*et110;
et111 = t1179-t1618+t1105.*(t485+t7.*(t53-t132));
et112 = (t1901+t1906+t1974-t1975+t1368.*(t485+t7.*(t53-t132)).*7.950000000000001e-3+t1383.*(t485+t7.*(t53-t132)).*2.2e-4)./2.0;
t2627 = et111.*et112;
t2629 = t2035.*(t1901+t1906+t1974-t1975+t1368.*(t485+t7.*(t53-t132)).*7.950000000000001e-3+t1383.*(t485+t7.*(t53-t132)).*2.2e-4).*(-1.0./2.0);
t2630 = (t2035.*(t1901+t1906+t1974-t1975+t1368.*(t485+t7.*(t53-t132)).*7.950000000000001e-3+t1383.*(t485+t7.*(t53-t132)).*2.2e-4))./2.0;
t2631 = t2049.*(t1896+t1903+t1976-t1977+t1368.*(t485+t7.*(t53-t132)).*2.2e-4+t1383.*(t485+t7.*(t53-t132)).*1.089e-2).*(-1.0./2.0);
et113 = (-t1614+t1626+t452.*(t515+t15.*(t57-t165))).*(t1896+t1903+t1976-t1977+t1368.*(t485+t7.*(t53-t132)).*2.2e-4+t1383.*(t485+t7.*(t53-t132)).*1.089e-2);
et114 = 1.0./2.0;
t2632 = et113.*et114;
t2634 = t2051.*(t1896+t1903+t1976-t1977+t1368.*(t485+t7.*(t53-t132)).*2.2e-4+t1383.*(t485+t7.*(t53-t132)).*1.089e-2).*(-1.0./2.0);
t2637 = t2084.*(t1896+t1903+t1976-t1977+t1368.*(t485+t7.*(t53-t132)).*2.2e-4+t1383.*(t485+t7.*(t53-t132)).*1.089e-2).*(-1.0./2.0);
t2638 = (t2084.*(t1896+t1903+t1976-t1977+t1368.*(t485+t7.*(t53-t132)).*2.2e-4+t1383.*(t485+t7.*(t53-t132)).*1.089e-2))./2.0;
et115 = -t1766+t396.*(t515+t15.*(t57-t165))+t1359.*(t485+t7.*(t53-t132));
et116 = (t1901+t1906+t1974-t1975+t1368.*(t485+t7.*(t53-t132)).*7.950000000000001e-3+t1383.*(t485+t7.*(t53-t132)).*2.2e-4)./2.0;
t2639 = et115.*et116;
t2641 = t2088.*(t1893+t1904+t1980-t1981+t1368.*(t485+t7.*(t53-t132)).*2.900000000000001e-4+t1383.*(t485+t7.*(t53-t132)).*2.9e-4).*(-1.0./2.0);
t2642 = (t2088.*(t1893+t1904+t1980-t1981+t1368.*(t485+t7.*(t53-t132)).*2.900000000000001e-4+t1383.*(t485+t7.*(t53-t132)).*2.9e-4))./2.0;
t2647 = t2113.*(t1893+t1904+t1980-t1981+t1368.*(t485+t7.*(t53-t132)).*2.900000000000001e-4+t1383.*(t485+t7.*(t53-t132)).*2.9e-4).*(-1.0./2.0);
t2648 = (t2113.*(t1893+t1904+t1980-t1981+t1368.*(t485+t7.*(t53-t132)).*2.900000000000001e-4+t1383.*(t485+t7.*(t53-t132)).*2.9e-4))./2.0;
t2649 = t2120.*(t1893+t1904+t1980-t1981+t1368.*(t485+t7.*(t53-t132)).*2.900000000000001e-4+t1383.*(t485+t7.*(t53-t132)).*2.9e-4).*(-1.0./2.0);
t2650 = t2121.*(t1893+t1904+t1980-t1981+t1368.*(t485+t7.*(t53-t132)).*2.900000000000001e-4+t1383.*(t485+t7.*(t53-t132)).*2.9e-4).*(-1.0./2.0);
et117 = t1560-t1637-t1754+t1857+t1879-t1927-t1943+t1060.*(t485+t7.*(t53-t132)).*7.950000000000001e-3;
et118 = t888.*(t257+t15.*(t273+t14.*(t51-t155))).*7.950000000000001e-3;
t2651 = t1768.*(et117+et118).*(-1.0./2.0);
et119 = t1780-t1790+t889.*(t8.*(t57-t165)+t15.*(t136-t246));
et120 = (t1893+t1904+t1980-t1981+t1368.*(t485+t7.*(t53-t132)).*2.900000000000001e-4+t1383.*(t485+t7.*(t53-t132)).*2.9e-4)./2.0;
t2652 = et119.*et120;
et121 = -t1595+t1607+t1828+t1851-t1940-t1955+t675.*(t8.*(t57-t165)+t15.*(t136-t246)).*2.900000000000001e-4+t14.*t1383.*(t129+t13.*(t51-t155)).*2.2e-4;
et122 = t14.*t1359.*(t156-t236).*2.2e-4;
t2654 = t1768.*(et121+et122).*(-1.0./2.0);
et123 = -t1595+t1607+t1828+t1851-t1940-t1955+t675.*(t8.*(t57-t165)+t15.*(t136-t246)).*2.900000000000001e-4+t14.*t1383.*(t129+t13.*(t51-t155)).*2.2e-4;
et124 = t14.*t1359.*(t156-t236).*2.2e-4;
t2656 = (t1768.*(et123+et124))./2.0;
et125 = t1984.*(t1550-t1633-t1760+t1856+t1878-t1931-t1948+t1060.*(t485+t7.*(t53-t132)).*2.900000000000001e-4+t888.*(t257+t15.*(t273+t14.*(t51-t155))).*2.900000000000001e-4);
et126 = -1.0./2.0;
t2672 = et125.*et126;
et127 = t1984.*(t1550-t1633-t1760+t1856+t1878-t1931-t1948+t1060.*(t485+t7.*(t53-t132)).*2.900000000000001e-4+t888.*(t257+t15.*(t273+t14.*(t51-t155))).*2.900000000000001e-4);
et128 = 1.0./2.0;
t2673 = et127.*et128;
et129 = -t1589+t1605+t1819+t1831-t1946-t1963+t675.*(t8.*(t57-t165)+t15.*(t136-t246)).*2.94e-3+t14.*t1383.*(t129+t13.*(t51-t155)).*2.9e-4;
et130 = t14.*t1359.*(t156-t236).*2.9e-4;
t2674 = t1984.*(et129+et130).*(-1.0./2.0);
et131 = t1752+t1383.*(t485+t7.*(t53-t132));
et132 = t1546-t1632-t1749+t1855+t1877-t1926-t1944+t1060.*(t485+t7.*(t53-t132)).*2.2e-4+t888.*(t257+t15.*(t273+t14.*(t51-t155))).*2.2e-4;
et133 = 1.0./2.0;
t2684 = et131.*et132.*et133;
et134 = t1560-t1637-t1754+t1857+t1879-t1927-t1943+t1060.*(t485+t7.*(t53-t132)).*7.950000000000001e-3;
et135 = t888.*(t257+t15.*(t273+t14.*(t51-t155))).*7.950000000000001e-3;
t2686 = ((et134+et135).*(t1743+t1368.*(t485+t7.*(t53-t132))))./2.0;
et136 = -t1584+t1604+t1823+t1839-t1942-t1957+t675.*(t8.*(t57-t165)+t15.*(t136-t246)).*2.9e-4+t14.*t1383.*(t129+t13.*(t51-t155)).*1.089e-2;
et137 = t14.*t1359.*(t156-t236).*1.089e-2;
t2688 = ((et136+et137).*(t1752+t1383.*(t485+t7.*(t53-t132))))./2.0;
et138 = -t1595+t1607+t1828+t1851-t1940-t1955+t675.*(t8.*(t57-t165)+t15.*(t136-t246)).*2.900000000000001e-4+t14.*t1383.*(t129+t13.*(t51-t155)).*2.2e-4;
et139 = t14.*t1359.*(t156-t236).*2.2e-4;
t2689 = ((et138+et139).*(t1743+t1368.*(t485+t7.*(t53-t132))))./2.0;
et140 = -t1595+t1607+t1828+t1851-t1940-t1955+t675.*(t8.*(t57-t165)+t15.*(t136-t246)).*2.900000000000001e-4+t14.*t1383.*(t129+t13.*(t51-t155)).*2.2e-4;
et141 = t14.*t1359.*(t156-t236).*2.2e-4;
t2692 = ((et140+et141).*(t1120+t1060.*(t485+t7.*(t53-t132))+t888.*(t257+t15.*(t273+t14.*(t51-t155)))))./2.0;
et142 = t1560-t1637-t1754+t1857+t1879-t1927-t1943+t1060.*(t485+t7.*(t53-t132)).*7.950000000000001e-3;
et143 = t888.*(t257+t15.*(t273+t14.*(t51-t155))).*7.950000000000001e-3;
t2698 = t2032.*(et142+et143).*(-1.0./2.0);
et144 = t1203+t14.*t1383.*(t129+t13.*(t51-t155))+t14.*t1359.*(t156-t236);
et145 = t1546-t1632-t1749+t1855+t1877-t1926-t1944+t1060.*(t485+t7.*(t53-t132)).*2.2e-4+t888.*(t257+t15.*(t273+t14.*(t51-t155))).*2.2e-4;
et146 = 1.0./2.0;
t2699 = et144.*et145.*et146;
et147 = t1560-t1637-t1754+t1857+t1879-t1927-t1943+t1060.*(t485+t7.*(t53-t132)).*7.950000000000001e-3;
et148 = t888.*(t257+t15.*(t273+t14.*(t51-t155))).*7.950000000000001e-3;
t2701 = ((et147+et148).*(t1179-t1618+t1105.*(t485+t7.*(t53-t132))))./2.0;
et149 = t1560-t1637-t1754+t1857+t1879-t1927-t1943+t1060.*(t485+t7.*(t53-t132)).*7.950000000000001e-3;
et150 = t888.*(t257+t15.*(t273+t14.*(t51-t155))).*7.950000000000001e-3;
t2702 = t2035.*(et149+et150).*(-1.0./2.0);
et151 = -t1595+t1607+t1828+t1851-t1940-t1955+t675.*(t8.*(t57-t165)+t15.*(t136-t246)).*2.900000000000001e-4+t14.*t1383.*(t129+t13.*(t51-t155)).*2.2e-4;
et152 = t14.*t1359.*(t156-t236).*2.2e-4;
t2703 = t2032.*(et151+et152).*(-1.0./2.0);
et153 = -t1595+t1607+t1828+t1851-t1940-t1955+t675.*(t8.*(t57-t165)+t15.*(t136-t246)).*2.900000000000001e-4+t14.*t1383.*(t129+t13.*(t51-t155)).*2.2e-4;
et154 = t14.*t1359.*(t156-t236).*2.2e-4;
t2704 = (t2032.*(et153+et154))./2.0;
et155 = -t1595+t1607+t1828+t1851-t1940-t1955+t675.*(t8.*(t57-t165)+t15.*(t136-t246)).*2.900000000000001e-4+t14.*t1383.*(t129+t13.*(t51-t155)).*2.2e-4;
et156 = t14.*t1359.*(t156-t236).*2.2e-4;
t2705 = t2035.*(et155+et156).*(-1.0./2.0);
et157 = -t1595+t1607+t1828+t1851-t1940-t1955+t675.*(t8.*(t57-t165)+t15.*(t136-t246)).*2.900000000000001e-4+t14.*t1383.*(t129+t13.*(t51-t155)).*2.2e-4;
et158 = t14.*t1359.*(t156-t236).*2.2e-4;
t2706 = (t2035.*(et157+et158))./2.0;
et159 = t2049.*(t1546-t1632-t1749+t1855+t1877-t1926-t1944+t1060.*(t485+t7.*(t53-t132)).*2.2e-4+t888.*(t257+t15.*(t273+t14.*(t51-t155))).*2.2e-4);
et160 = -1.0./2.0;
t2709 = et159.*et160;
et161 = t2049.*(t1546-t1632-t1749+t1855+t1877-t1926-t1944+t1060.*(t485+t7.*(t53-t132)).*2.2e-4+t888.*(t257+t15.*(t273+t14.*(t51-t155))).*2.2e-4);
et162 = 1.0./2.0;
t2710 = et161.*et162;
et163 = -t1614+t1626+t452.*(t515+t15.*(t57-t165));
et164 = t1546-t1632-t1749+t1855+t1877-t1926-t1944+t1060.*(t485+t7.*(t53-t132)).*2.2e-4+t888.*(t257+t15.*(t273+t14.*(t51-t155))).*2.2e-4;
et165 = 1.0./2.0;
t2711 = et163.*et164.*et165;
et166 = -t1584+t1604+t1823+t1839-t1942-t1957+t675.*(t8.*(t57-t165)+t15.*(t136-t246)).*2.9e-4+t14.*t1383.*(t129+t13.*(t51-t155)).*1.089e-2;
et167 = t14.*t1359.*(t156-t236).*1.089e-2;
t2713 = t2049.*(et166+et167).*(-1.0./2.0);
et168 = -t1584+t1604+t1823+t1839-t1942-t1957+t675.*(t8.*(t57-t165)+t15.*(t136-t246)).*2.9e-4+t14.*t1383.*(t129+t13.*(t51-t155)).*1.089e-2;
et169 = t14.*t1359.*(t156-t236).*1.089e-2;
t2719 = ((et168+et169).*(-t1614+t1626+t452.*(t515+t15.*(t57-t165))))./2.0;
et170 = -t1584+t1604+t1823+t1839-t1942-t1957+t675.*(t8.*(t57-t165)+t15.*(t136-t246)).*2.9e-4+t14.*t1383.*(t129+t13.*(t51-t155)).*1.089e-2;
et171 = t14.*t1359.*(t156-t236).*1.089e-2;
t2720 = t2051.*(et170+et171).*(-1.0./2.0);
et172 = t2084.*(t1546-t1632-t1749+t1855+t1877-t1926-t1944+t1060.*(t485+t7.*(t53-t132)).*2.2e-4+t888.*(t257+t15.*(t273+t14.*(t51-t155))).*2.2e-4);
et173 = -1.0./2.0;
t2735 = et172.*et173;
et174 = t1560-t1637-t1754+t1857+t1879-t1927-t1943+t1060.*(t485+t7.*(t53-t132)).*7.950000000000001e-3;
et175 = t888.*(t257+t15.*(t273+t14.*(t51-t155))).*7.950000000000001e-3;
t2737 = ((et174+et175).*(-t1766+t396.*(t515+t15.*(t57-t165))+t1359.*(t485+t7.*(t53-t132))))./2.0;
et176 = -t1584+t1604+t1823+t1839-t1942-t1957+t675.*(t8.*(t57-t165)+t15.*(t136-t246)).*2.9e-4+t14.*t1383.*(t129+t13.*(t51-t155)).*1.089e-2;
et177 = t14.*t1359.*(t156-t236).*1.089e-2;
t2738 = t2084.*(et176+et177).*(-1.0./2.0);
et178 = -t1584+t1604+t1823+t1839-t1942-t1957+t675.*(t8.*(t57-t165)+t15.*(t136-t246)).*2.9e-4+t14.*t1383.*(t129+t13.*(t51-t155)).*1.089e-2;
et179 = t14.*t1359.*(t156-t236).*1.089e-2;
t2739 = (t2084.*(et178+et179))./2.0;
et180 = t2088.*(t1550-t1633-t1760+t1856+t1878-t1931-t1948+t1060.*(t485+t7.*(t53-t132)).*2.900000000000001e-4+t888.*(t257+t15.*(t273+t14.*(t51-t155))).*2.900000000000001e-4);
et181 = -1.0./2.0;
t2740 = et180.*et181;
et182 = -t1595+t1607+t1828+t1851-t1940-t1955+t675.*(t8.*(t57-t165)+t15.*(t136-t246)).*2.900000000000001e-4+t14.*t1383.*(t129+t13.*(t51-t155)).*2.2e-4;
et183 = t14.*t1359.*(t156-t236).*2.2e-4;
t2741 = ((et182+et183).*(-t1766+t396.*(t515+t15.*(t57-t165))+t1359.*(t485+t7.*(t53-t132))))./2.0;
et184 = -t1589+t1605+t1819+t1831-t1946-t1963+t675.*(t8.*(t57-t165)+t15.*(t136-t246)).*2.94e-3+t14.*t1383.*(t129+t13.*(t51-t155)).*2.9e-4;
et185 = t14.*t1359.*(t156-t236).*2.9e-4;
t2744 = t2088.*(et184+et185).*(-1.0./2.0);
et186 = -t1589+t1605+t1819+t1831-t1946-t1963+t675.*(t8.*(t57-t165)+t15.*(t136-t246)).*2.94e-3+t14.*t1383.*(t129+t13.*(t51-t155)).*2.9e-4;
et187 = t14.*t1359.*(t156-t236).*2.9e-4;
t2746 = (t2088.*(et186+et187))./2.0;
et188 = -t1589+t1605+t1819+t1831-t1946-t1963+t675.*(t8.*(t57-t165)+t15.*(t136-t246)).*2.94e-3+t14.*t1383.*(t129+t13.*(t51-t155)).*2.9e-4;
et189 = t14.*t1359.*(t156-t236).*2.9e-4;
t2757 = t2113.*(et188+et189).*(-1.0./2.0);
et190 = -t1589+t1605+t1819+t1831-t1946-t1963+t675.*(t8.*(t57-t165)+t15.*(t136-t246)).*2.94e-3+t14.*t1383.*(t129+t13.*(t51-t155)).*2.9e-4;
et191 = t14.*t1359.*(t156-t236).*2.9e-4;
t2758 = (t2113.*(et190+et191))./2.0;
et192 = t2120.*(t1550-t1633-t1760+t1856+t1878-t1931-t1948+t1060.*(t485+t7.*(t53-t132)).*2.900000000000001e-4+t888.*(t257+t15.*(t273+t14.*(t51-t155))).*2.900000000000001e-4);
et193 = -1.0./2.0;
t2759 = et192.*et193;
et194 = t2121.*(t1550-t1633-t1760+t1856+t1878-t1931-t1948+t1060.*(t485+t7.*(t53-t132)).*2.900000000000001e-4+t888.*(t257+t15.*(t273+t14.*(t51-t155))).*2.900000000000001e-4);
et195 = -1.0./2.0;
t2760 = et194.*et195;
et196 = t2120.*(t1550-t1633-t1760+t1856+t1878-t1931-t1948+t1060.*(t485+t7.*(t53-t132)).*2.900000000000001e-4+t888.*(t257+t15.*(t273+t14.*(t51-t155))).*2.900000000000001e-4);
et197 = 1.0./2.0;
t2761 = et196.*et197;
et198 = t2121.*(t1550-t1633-t1760+t1856+t1878-t1931-t1948+t1060.*(t485+t7.*(t53-t132)).*2.900000000000001e-4+t888.*(t257+t15.*(t273+t14.*(t51-t155))).*2.900000000000001e-4);
et199 = 1.0./2.0;
t2762 = et198.*et199;
et200 = -t1589+t1605+t1819+t1831-t1946-t1963+t675.*(t8.*(t57-t165)+t15.*(t136-t246)).*2.94e-3+t14.*t1383.*(t129+t13.*(t51-t155)).*2.9e-4;
et201 = t14.*t1359.*(t156-t236).*2.9e-4;
t2763 = t2121.*(et200+et201).*(-1.0./2.0);
et202 = t1780-t1790+t889.*(t8.*(t57-t165)+t15.*(t136-t246));
et203 = t1550-t1633-t1760+t1856+t1878-t1931-t1948+t1060.*(t485+t7.*(t53-t132)).*2.900000000000001e-4+t888.*(t257+t15.*(t273+t14.*(t51-t155))).*2.900000000000001e-4;
et204 = 1.0./2.0;
t2764 = et202.*et203.*et204;
et205 = -t1589+t1605+t1819+t1831-t1946-t1963+t675.*(t8.*(t57-t165)+t15.*(t136-t246)).*2.94e-3+t14.*t1383.*(t129+t13.*(t51-t155)).*2.9e-4;
et206 = t14.*t1359.*(t156-t236).*2.9e-4;
t2767 = ((et205+et206).*(t1780-t1790+t889.*(t8.*(t57-t165)+t15.*(t136-t246))))./2.0;
t2285 = -t2283;
t2293 = -t2291;
t2299 = -t2298;
t2322 = -t2321;
t2354 = -t2352;
t2367 = -t2365;
t2384 = -t2382;
t2386 = -t2385;
t2388 = -t2387;
t2393 = -t2392;
t2405 = -t2404;
t2438 = -t2437;
t2449 = -t2448;
t2455 = t1500+t1678+t1712+t1740+t1897+t1921;
t2457 = t1502+t1689+t1714+t1733+t1902+t1924;
t2458 = t1512+t1682+t1722+t1746+t1894+t1923;
t2487 = -t2486;
t2489 = -t2488;
t2494 = -t2493;
t2509 = -t2508;
t2514 = -t2513;
t2519 = -t2518;
t2521 = -t2520;
t2532 = t1899+t1905+t1909+t1915+t1977+t1979;
t2533 = t1908+t1911+t1912+t1918+t1975+t1978;
t2534 = t1898+t1900+t1910+t1916+t1981+t1982;
t2543 = -t2540;
t2569 = -t2568;
t2578 = t2069.*(t1507+t1719+t1741-t1923+t396.*(t515+t15.*(t57-t165)).*2.900000000000001e-4+t1359.*(t485+t7.*(t53-t132)).*2.900000000000001e-4).*(-1.0./2.0);
t2588 = -t2585;
t2594 = -t2593;
t2596 = -t2595;
t2610 = t1555+t1632+t1749+t1806+t1817+t1859+t1880+t1926+t1944;
t2611 = t1565+t1637+t1754+t1809+t1825+t1861+t1882+t1927+t1943;
t2612 = t1556+t1633+t1760+t1807+t1816+t1860+t1881+t1931+t1948;
t2619 = t1659+t1690+t1795+t1811+t1813+t1832+t1865+t1936+t1939;
t2620 = t1669+t1695+t1794+t1814+t1822+t1835+t1864+t1934+t1941;
t2621 = t1653+t1691+t1798+t1812+t1815+t1833+t1866+t1938+t1947;
t2623 = -t2622;
t2628 = -t2627;
t2633 = -t2632;
t2635 = (t1984.*t2605)./2.0;
t2640 = -t2639;
t2643 = t2604.*(t1752+t1383.*(t485+t7.*(t53-t132))).*(-1.0./2.0);
t2644 = (t2604.*(t1752+t1383.*(t485+t7.*(t53-t132))))./2.0;
t2645 = t2606.*(t1743+t1368.*(t485+t7.*(t53-t132))).*(-1.0./2.0);
t2646 = (t2606.*(t1743+t1368.*(t485+t7.*(t53-t132))))./2.0;
t2653 = t2606.*(t1120+t1060.*(t485+t7.*(t53-t132))+t888.*(t257+t15.*(t273+t14.*(t51-t155)))).*(-1.0./2.0);
t2655 = -t2652;
t2657 = (t2032.*t2606)./2.0;
t2658 = t2604.*(t1203+t14.*t1383.*(t129+t13.*(t51-t155))+t14.*t1359.*(t156-t236)).*(-1.0./2.0);
t2659 = (t2604.*(t1203+t14.*t1383.*(t129+t13.*(t51-t155))+t14.*t1359.*(t156-t236)))./2.0;
t2660 = t2606.*(t1179-t1618+t1105.*(t485+t7.*(t53-t132))).*(-1.0./2.0);
t2661 = (t2035.*t2606)./2.0;
t2662 = (t1768.*t2618)./2.0;
t2665 = (t2049.*t2604)./2.0;
t2667 = t2604.*(-t1614+t1626+t452.*(t515+t15.*(t57-t165))).*(-1.0./2.0);
t2668 = (t2051.*t2604)./2.0;
t2670 = (t2069.*t2605)./2.0;
t2671 = t2606.*(-t1766+t396.*(t515+t15.*(t57-t165))+t1359.*(t485+t7.*(t53-t132))).*(-1.0./2.0);
t2675 = (t2113.*t2605)./2.0;
t2676 = (t2120.*t2605)./2.0;
t2678 = (t2121.*t2605)./2.0;
t2679 = (t1984.*t2617)./2.0;
t2681 = t2605.*(t1780-t1790+t889.*(t8.*(t57-t165)+t15.*(t136-t246))).*(-1.0./2.0);
t2685 = -t2684;
t2687 = -t2686;
t2690 = t2616.*(t1752+t1383.*(t485+t7.*(t53-t132))).*(-1.0./2.0);
t2691 = t2618.*(t1743+t1368.*(t485+t7.*(t53-t132))).*(-1.0./2.0);
t2693 = -t2692;
t2700 = -t2699;
t2707 = t2618.*(t1120+t1060.*(t485+t7.*(t53-t132))+t888.*(t257+t15.*(t273+t14.*(t51-t155)))).*(-1.0./2.0);
t2708 = (t2618.*(t1120+t1060.*(t485+t7.*(t53-t132))+t888.*(t257+t15.*(t273+t14.*(t51-t155)))))./2.0;
t2714 = t2616.*(t1203+t14.*t1383.*(t129+t13.*(t51-t155))+t14.*t1359.*(t156-t236)).*(-1.0./2.0);
t2715 = t2618.*(t1179-t1618+t1105.*(t485+t7.*(t53-t132))).*(-1.0./2.0);
t2716 = (t2618.*(t1179-t1618+t1105.*(t485+t7.*(t53-t132))))./2.0;
t2717 = (t2035.*t2618)./2.0;
t2721 = -t2719;
t2726 = t2616.*(-t1614+t1626+t452.*(t515+t15.*(t57-t165))).*(-1.0./2.0);
t2727 = (t2051.*t2616)./2.0;
t2728 = (t2616.*(-t1614+t1626+t452.*(t515+t15.*(t57-t165))))./2.0;
et207 = t2069.*(t1550-t1633-t1760+t1856+t1878-t1931-t1948+t1060.*(t485+t7.*(t53-t132)).*2.900000000000001e-4+t888.*(t257+t15.*(t273+t14.*(t51-t155))).*2.900000000000001e-4);
et208 = -1.0./2.0;
t2729 = et207.*et208;
et209 = -t1589+t1605+t1819+t1831-t1946-t1963+t675.*(t8.*(t57-t165)+t15.*(t136-t246)).*2.94e-3+t14.*t1383.*(t129+t13.*(t51-t155)).*2.9e-4;
et210 = t14.*t1359.*(t156-t236).*2.9e-4;
t2730 = t2069.*(et209+et210).*(-1.0./2.0);
et211 = -t1589+t1605+t1819+t1831-t1946-t1963+t675.*(t8.*(t57-t165)+t15.*(t136-t246)).*2.94e-3+t14.*t1383.*(t129+t13.*(t51-t155)).*2.9e-4;
et212 = t14.*t1359.*(t156-t236).*2.9e-4;
t2731 = (t2069.*(et211+et212))./2.0;
t2742 = -t2741;
t2743 = (t2069.*t2617)./2.0;
t2748 = (t2084.*t2616)./2.0;
t2750 = t2618.*(-t1766+t396.*(t515+t15.*(t57-t165))+t1359.*(t485+t7.*(t53-t132))).*(-1.0./2.0);
t2751 = (t2618.*(-t1766+t396.*(t515+t15.*(t57-t165))+t1359.*(t485+t7.*(t53-t132))))./2.0;
t2752 = (t2088.*t2617)./2.0;
t2765 = (t2113.*t2617)./2.0;
t2768 = -t2767;
t2769 = (t2120.*t2617)./2.0;
t2771 = t2617.*(t1780-t1790+t889.*(t8.*(t57-t165)+t15.*(t136-t246))).*(-1.0./2.0);
t2772 = (t2617.*(t1780-t1790+t889.*(t8.*(t57-t165)+t15.*(t136-t246))))./2.0;
t2780 = t2195+t2286+t2302+t2528+t2562+t2598+t2673+t2737;
t2636 = -t2635;
t2663 = -t2662;
t2664 = (t1768.*t2620)./2.0;
t2666 = -t2665;
t2669 = -t2668;
t2677 = -t2676;
t2680 = -t2678;
t2682 = (t1984.*t2621)./2.0;
t2694 = t2619.*(t1752+t1383.*(t485+t7.*(t53-t132))).*(-1.0./2.0);
t2695 = (t2619.*(t1752+t1383.*(t485+t7.*(t53-t132))))./2.0;
t2696 = t2620.*(t1743+t1368.*(t485+t7.*(t53-t132))).*(-1.0./2.0);
t2697 = (t2620.*(t1743+t1368.*(t485+t7.*(t53-t132))))./2.0;
t2712 = t2620.*(t1120+t1060.*(t485+t7.*(t53-t132))+t888.*(t257+t15.*(t273+t14.*(t51-t155)))).*(-1.0./2.0);
t2718 = -t2717;
t2722 = (t2032.*t2620)./2.0;
t2723 = t2619.*(t1203+t14.*t1383.*(t129+t13.*(t51-t155))+t14.*t1359.*(t156-t236)).*(-1.0./2.0);
t2724 = (t2619.*(t1203+t14.*t1383.*(t129+t13.*(t51-t155))+t14.*t1359.*(t156-t236)))./2.0;
t2725 = t2620.*(t1179-t1618+t1105.*(t485+t7.*(t53-t132))).*(-1.0./2.0);
t2732 = (t2049.*t2619)./2.0;
t2734 = (t2051.*t2619)./2.0;
t2745 = -t2743;
t2747 = (t2069.*t2621)./2.0;
t2749 = -t2748;
t2753 = -t2752;
t2754 = (t2084.*t2619)./2.0;
t2755 = t2620.*(-t1766+t396.*(t515+t15.*(t57-t165))+t1359.*(t485+t7.*(t53-t132))).*(-1.0./2.0);
t2756 = (t2088.*t2621)./2.0;
t2766 = -t2765;
t2770 = (t2113.*t2621)./2.0;
t2773 = (t2120.*t2621)./2.0;
t2774 = (t2121.*t2621)./2.0;
t2777 = t2359+t2360+t2519+t2521+t2578+t2609+t2640;
t2779 = t2153+t2262+t2268+t2543+t2544+t2601+t2674+t2742;
t2781 = t2182+t2304+t2305+t2539+t2557+t2602+t2679+t2751;
t2783 = t2218+t2222+t2346+t2349+t2395+t2399+t2432+t2464+t2485+t2608+t2638+t2642+t2644+t2646+t2670;
t2788 = t2115+t2117+t2204+t2206+t2236+t2256+t2274+t2316+t2371+t2373+t2374+t2460+t2480+t2487+t2494+t2495+t2510+t2626+t2628+t2649+t2688+t2689+t2731;
t2789 = t1998+t2031+t2039+t2083+t2145+t2151+t2215+t2228+t2253+t2276+t2310+t2328+t2383+t2431+t2496+t2499+t2504+t2522+t2567+t2573+t2693+t2700+t2701+t2720+t2758+t2761;
t2790 = t2018+t2060+t2064+t2096+t2168+t2169+t2197+t2241+t2260+t2295+t2325+t2329+t2410+t2456+t2498+t2501+t2509+t2516+t2575+t2579+t2704+t2713+t2714+t2716+t2763+t2769;
t2792 = t2062+t2063+t2104+t2106+t2150+t2154+t2188+t2202+t2226+t2248+t2249+t2306+t2356+t2358+t2386+t2388+t2394+t2403+t2411+t2466+t2468+t2490+t2525+t2527+t2563+t2623+t2634+t2648+t2685+t2687+t2729;
t2683 = -t2682;
t2733 = -t2732;
t2736 = -t2734;
t2775 = -t2773;
t2776 = -t2774;
t2778 = t2137+t2242+t2250+t2483+t2587+t2589+t2636+t2671;
t2784 = t2045+t2124+t2132+t2146+t2255+t2265+t2372+t2429+t2438+t2492+t2511+t2656+t2659+t2660+t2677+t2739+t2746;
t2785 = t2091+t2149+t2158+t2190+t2278+t2293+t2405+t2414+t2452+t2512+t2571+t2651+t2653+t2669+t2675+t2735+t2740;
t2786 = t2102+t2172+t2178+t2180+t2294+t2297+t2408+t2422+t2449+t2514+t2577+t2657+t2663+t2666+t2680+t2749+t2753;
M = ft_6({q1,q2,t10,t1020,t1033,t1034,t1039,t1060,t1066,t1079,t1080,t1090,t1094,t1095,t1097,t1105,t1107,t1116,t1117,t1119,t112,t1120,t1124,t1125,t1131,t1132,t1136,t1140,t1146,t1149,t1151,t1155,t1159,t1168,t1179,t1182,t1183,t1189,t119,t1194,t1197,t1198,t120,t1203,t1204,t121,t1213,t122,t1222,t1229,t1232,t1250,t1255,t1269,t1272,t1284,t129,t1292,t1293,t13,t130,t1300,t1312,t132,t1324,t1327,t1333,t1337,t1338,t1340,t1341,t1342,t1359,t136,t1364,t1365,t1366,t1368,t1375,t1383,t1394,t1396,t1398,t14,t1403,t1404,t1410,t1414,t1417,t1419,t1425,t143,t1432,t1465,t1475,t1486,t1499,t15,t1501,t1504,t1505,t1507,t1518,t1523,t1526,t1529,t153,t1530,t1535,t1537,t1542,t1546,t155,t1550,t1552,t156,t1560,t1568,t1569,t1575,t1584,t1589,t1593,t1595,t16,t1601,t1603,t1604,t1605,t1606,t1607,t1614,t1618,t1621,t1625,t1626,t1627,t1629,t1632,t1633,t1637,t164,t1645,t1648,t165,t1658,t1662,t1665,t167,t1671,t1687,t1697,t1699,t17,t170,t1704,t1707,t1709,t1710,t1711,t1715,t1719,t172,t1726,t173,t1731,t1736,t1738,t1741,t1743,t1749,t1752,t1754,t1757,t1760,t1766,t1768,t1769,t1771,t1772,t1773,t1776,t1777,t1780,t1782,t1783,t1784,t1785,t1789,t1790,t1797,t18,t180,t1802,t1803,t1804,t1805,t1808,t1810,t1819,t1823,t1826,t1828,t1831,t1839,t1851,t1855,t1856,t1857,t1867,t1877,t1878,t1879,t1883,t1884,t1885,t1893,t1896,t1901,t1903,t1904,t1906,t191,t1919,t1923,t1924,t1926,t1927,t1929,t1930,t1931,t1935,t1940,t1942,t1943,t1944,t1945,t1946,t1948,t1949,t1952,t1953,t1954,t1955,t1957,t1960,t1961,t1963,t1964,t1965,t1966,t1967,t1969,t1970,t1972,t1973,t1974,t1975,t1976,t1977,t1980,t1981,t1983,t1984,t1985,t1986,t1987,t1990,t1991,t1992,t1993,t1996,t1997,t1999,t2000,t2001,t2002,t2003,t2004,t2005,t2006,t2007,t2008,t2009,t2011,t2013,t2016,t2017,t2019,t2021,t2024,t2025,t2027,t2029,t203,t2032,t2033,t2035,t2036,t2041,t2043,t2047,t2048,t2049,t205,t2051,t2054,t2055,t2056,t2057,t2059,t2065,t2066,t2067,t2068,t2069,t2070,t2072,t2073,t2075,t2077,t2079,t2080,t2081,t2082,t2084,t2088,t2089,t2090,t2093,t2094,t2095,t2098,t210,t2101,t2107,t2109,t2111,t2112,t2113,t2114,t2118,t2120,t2121,t2122,t2126,t2128,t2129,t2131,t2133,t2134,t2135,t2136,t2139,t2141,t2142,t2148,t2152,t2156,t2161,t2162,t2164,t2166,t2170,t2174,t2175,t2176,t2183,t2184,t2187,t2189,t2191,t2193,t2194,t2201,t2203,t2205,t2208,t2210,t2211,t2212,t2214,t2216,t2221,t2223,t2225,t2229,t223,t2231,t2232,t2234,t2235,t2237,t2239,t2244,t2246,t225,t2254,t2258,t2259,t2261,t2263,t2264,t2266,t2267,t2269,t227,t2271,t2272,t2273,t228,t2281,t2285,t2287,t2288,t2289,t2290,t2299,t2309,t231,t2311,t2313,t2314,t2315,t2318,t2320,t2322,t2323,t2331,t2332,t2334,t2335,t2337,t2339,t2340,t2341,t2343,t2344,t2345,t2347,t2348,t2351,t2354,t2355,t236,t2361,t2362,t2363,t2364,t2366,t2367,t2370,t2376,t2377,t2378,t2379,t2380,t2384,t2390,t2391,t2393,t2397,t2401,t2406,t2409,t2413,t2415,t2416,t2418,t2419,t2421,t2423,t2425,t2427,t2430,t2434,t2435,t2436,t2439,t2440,t2441,t2442,t2443,t2444,t2445,t2446,t2447,t2450,t2451,t2453,t2454,t2459,t246,t2461,t2462,t2467,t2469,t2472,t2473,t2475,t2476,t2478,t2479,t2489,t2491,t2505,t2506,t2507,t2517,t252,t2523,t2530,t2531,t2536,t2537,t2541,t2542,t2545,t2546,t2549,t2550,t2551,t2553,t2554,t2555,t2558,t2559,t2560,t2565,t2569,t257,t2576,t2581,t2583,t2586,t2588,t2590,t2592,t2594,t2596,t2597,t2603,t2604,t2605,t2606,t2616,t2617,t2618,t2619,t2620,t2621,t2625,t2630,t2631,t2633,t2650,t2655,t2661,t2664,t2667,t2681,t2683,t2690,t2691,t2695,t2697,t2698,t2702,t2706,t2708,t2710,t2711,t2712,t2718,t2721,t2722,t2724,t2725,t2727,t2728,t273,t2733,t2736,t2745,t2747,t2754,t2755,t2756,t2762,t2764,t2766,t2768,t277,t2770,t2772,t2775,t2776,t2777,t2778,t2779,t2780,t2781,t2783,t2784,t2785,t2786,t2788,t2789,t2790,t2792,t300,t308,t31,t311,t312,t313,t314,t315,t32,t328,t33,t333,t342,t346,t36,t395,t396,t397,t451,t452,t455,t470,t485,t5,t500,t51,t515,t53,t533,t544,t55,t565,t57,t580,t6,t614,t639,t648,t654,t655,t66,t671,t673,t675,t679,t68,t7,t703,t710,t711,t717,t725,t726,t727,t748,t75,t765,t769,t770,t773,t788,t795,t8,t822,t826,t836,t854,t856,t865,t87,t873,t888,t889,t890,t896,t9,t902,t909,t910,t914,t929,t930,t933,t938,t942,t944,t969,t977,t979,t98,t980});
end
function M = ft_6(ct)
q1 = ct{1};
q2 = ct{2};
t10 = ct{3};
t1020 = ct{4};
t1033 = ct{5};
t1034 = ct{6};
t1039 = ct{7};
t1060 = ct{8};
t1066 = ct{9};
t1079 = ct{10};
t1080 = ct{11};
t1090 = ct{12};
t1094 = ct{13};
t1095 = ct{14};
t1097 = ct{15};
t1105 = ct{16};
t1107 = ct{17};
t1116 = ct{18};
t1117 = ct{19};
t1119 = ct{20};
t112 = ct{21};
t1120 = ct{22};
t1124 = ct{23};
t1125 = ct{24};
t1131 = ct{25};
t1132 = ct{26};
t1136 = ct{27};
t1140 = ct{28};
t1146 = ct{29};
t1149 = ct{30};
t1151 = ct{31};
t1155 = ct{32};
t1159 = ct{33};
t1168 = ct{34};
t1179 = ct{35};
t1182 = ct{36};
t1183 = ct{37};
t1189 = ct{38};
t119 = ct{39};
t1194 = ct{40};
t1197 = ct{41};
t1198 = ct{42};
t120 = ct{43};
t1203 = ct{44};
t1204 = ct{45};
t121 = ct{46};
t1213 = ct{47};
t122 = ct{48};
t1222 = ct{49};
t1229 = ct{50};
t1232 = ct{51};
t1250 = ct{52};
t1255 = ct{53};
t1269 = ct{54};
t1272 = ct{55};
t1284 = ct{56};
t129 = ct{57};
t1292 = ct{58};
t1293 = ct{59};
t13 = ct{60};
t130 = ct{61};
t1300 = ct{62};
t1312 = ct{63};
t132 = ct{64};
t1324 = ct{65};
t1327 = ct{66};
t1333 = ct{67};
t1337 = ct{68};
t1338 = ct{69};
t1340 = ct{70};
t1341 = ct{71};
t1342 = ct{72};
t1359 = ct{73};
t136 = ct{74};
t1364 = ct{75};
t1365 = ct{76};
t1366 = ct{77};
t1368 = ct{78};
t1375 = ct{79};
t1383 = ct{80};
t1394 = ct{81};
t1396 = ct{82};
t1398 = ct{83};
t14 = ct{84};
t1403 = ct{85};
t1404 = ct{86};
t1410 = ct{87};
t1414 = ct{88};
t1417 = ct{89};
t1419 = ct{90};
t1425 = ct{91};
t143 = ct{92};
t1432 = ct{93};
t1465 = ct{94};
t1475 = ct{95};
t1486 = ct{96};
t1499 = ct{97};
t15 = ct{98};
t1501 = ct{99};
t1504 = ct{100};
t1505 = ct{101};
t1507 = ct{102};
t1518 = ct{103};
t1523 = ct{104};
t1526 = ct{105};
t1529 = ct{106};
t153 = ct{107};
t1530 = ct{108};
t1535 = ct{109};
t1537 = ct{110};
t1542 = ct{111};
t1546 = ct{112};
t155 = ct{113};
t1550 = ct{114};
t1552 = ct{115};
t156 = ct{116};
t1560 = ct{117};
t1568 = ct{118};
t1569 = ct{119};
t1575 = ct{120};
t1584 = ct{121};
t1589 = ct{122};
t1593 = ct{123};
t1595 = ct{124};
t16 = ct{125};
t1601 = ct{126};
t1603 = ct{127};
t1604 = ct{128};
t1605 = ct{129};
t1606 = ct{130};
t1607 = ct{131};
t1614 = ct{132};
t1618 = ct{133};
t1621 = ct{134};
t1625 = ct{135};
t1626 = ct{136};
t1627 = ct{137};
t1629 = ct{138};
t1632 = ct{139};
t1633 = ct{140};
t1637 = ct{141};
t164 = ct{142};
t1645 = ct{143};
t1648 = ct{144};
t165 = ct{145};
t1658 = ct{146};
t1662 = ct{147};
t1665 = ct{148};
t167 = ct{149};
t1671 = ct{150};
t1687 = ct{151};
t1697 = ct{152};
t1699 = ct{153};
t17 = ct{154};
t170 = ct{155};
t1704 = ct{156};
t1707 = ct{157};
t1709 = ct{158};
t1710 = ct{159};
t1711 = ct{160};
t1715 = ct{161};
t1719 = ct{162};
t172 = ct{163};
t1726 = ct{164};
t173 = ct{165};
t1731 = ct{166};
t1736 = ct{167};
t1738 = ct{168};
t1741 = ct{169};
t1743 = ct{170};
t1749 = ct{171};
t1752 = ct{172};
t1754 = ct{173};
t1757 = ct{174};
t1760 = ct{175};
t1766 = ct{176};
t1768 = ct{177};
t1769 = ct{178};
t1771 = ct{179};
t1772 = ct{180};
t1773 = ct{181};
t1776 = ct{182};
t1777 = ct{183};
t1780 = ct{184};
t1782 = ct{185};
t1783 = ct{186};
t1784 = ct{187};
t1785 = ct{188};
t1789 = ct{189};
t1790 = ct{190};
t1797 = ct{191};
t18 = ct{192};
t180 = ct{193};
t1802 = ct{194};
t1803 = ct{195};
t1804 = ct{196};
t1805 = ct{197};
t1808 = ct{198};
t1810 = ct{199};
t1819 = ct{200};
t1823 = ct{201};
t1826 = ct{202};
t1828 = ct{203};
t1831 = ct{204};
t1839 = ct{205};
t1851 = ct{206};
t1855 = ct{207};
t1856 = ct{208};
t1857 = ct{209};
t1867 = ct{210};
t1877 = ct{211};
t1878 = ct{212};
t1879 = ct{213};
t1883 = ct{214};
t1884 = ct{215};
t1885 = ct{216};
t1893 = ct{217};
t1896 = ct{218};
t1901 = ct{219};
t1903 = ct{220};
t1904 = ct{221};
t1906 = ct{222};
t191 = ct{223};
t1919 = ct{224};
t1923 = ct{225};
t1924 = ct{226};
t1926 = ct{227};
t1927 = ct{228};
t1929 = ct{229};
t1930 = ct{230};
t1931 = ct{231};
t1935 = ct{232};
t1940 = ct{233};
t1942 = ct{234};
t1943 = ct{235};
t1944 = ct{236};
t1945 = ct{237};
t1946 = ct{238};
t1948 = ct{239};
t1949 = ct{240};
t1952 = ct{241};
t1953 = ct{242};
t1954 = ct{243};
t1955 = ct{244};
t1957 = ct{245};
t1960 = ct{246};
t1961 = ct{247};
t1963 = ct{248};
t1964 = ct{249};
t1965 = ct{250};
t1966 = ct{251};
t1967 = ct{252};
t1969 = ct{253};
t1970 = ct{254};
t1972 = ct{255};
t1973 = ct{256};
t1974 = ct{257};
t1975 = ct{258};
t1976 = ct{259};
t1977 = ct{260};
t1980 = ct{261};
t1981 = ct{262};
t1983 = ct{263};
t1984 = ct{264};
t1985 = ct{265};
t1986 = ct{266};
t1987 = ct{267};
t1990 = ct{268};
t1991 = ct{269};
t1992 = ct{270};
t1993 = ct{271};
t1996 = ct{272};
t1997 = ct{273};
t1999 = ct{274};
t2000 = ct{275};
t2001 = ct{276};
t2002 = ct{277};
t2003 = ct{278};
t2004 = ct{279};
t2005 = ct{280};
t2006 = ct{281};
t2007 = ct{282};
t2008 = ct{283};
t2009 = ct{284};
t2011 = ct{285};
t2013 = ct{286};
t2016 = ct{287};
t2017 = ct{288};
t2019 = ct{289};
t2021 = ct{290};
t2024 = ct{291};
t2025 = ct{292};
t2027 = ct{293};
t2029 = ct{294};
t203 = ct{295};
t2032 = ct{296};
t2033 = ct{297};
t2035 = ct{298};
t2036 = ct{299};
t2041 = ct{300};
t2043 = ct{301};
t2047 = ct{302};
t2048 = ct{303};
t2049 = ct{304};
t205 = ct{305};
t2051 = ct{306};
t2054 = ct{307};
t2055 = ct{308};
t2056 = ct{309};
t2057 = ct{310};
t2059 = ct{311};
t2065 = ct{312};
t2066 = ct{313};
t2067 = ct{314};
t2068 = ct{315};
t2069 = ct{316};
t2070 = ct{317};
t2072 = ct{318};
t2073 = ct{319};
t2075 = ct{320};
t2077 = ct{321};
t2079 = ct{322};
t2080 = ct{323};
t2081 = ct{324};
t2082 = ct{325};
t2084 = ct{326};
t2088 = ct{327};
t2089 = ct{328};
t2090 = ct{329};
t2093 = ct{330};
t2094 = ct{331};
t2095 = ct{332};
t2098 = ct{333};
t210 = ct{334};
t2101 = ct{335};
t2107 = ct{336};
t2109 = ct{337};
t2111 = ct{338};
t2112 = ct{339};
t2113 = ct{340};
t2114 = ct{341};
t2118 = ct{342};
t2120 = ct{343};
t2121 = ct{344};
t2122 = ct{345};
t2126 = ct{346};
t2128 = ct{347};
t2129 = ct{348};
t2131 = ct{349};
t2133 = ct{350};
t2134 = ct{351};
t2135 = ct{352};
t2136 = ct{353};
t2139 = ct{354};
t2141 = ct{355};
t2142 = ct{356};
t2148 = ct{357};
t2152 = ct{358};
t2156 = ct{359};
t2161 = ct{360};
t2162 = ct{361};
t2164 = ct{362};
t2166 = ct{363};
t2170 = ct{364};
t2174 = ct{365};
t2175 = ct{366};
t2176 = ct{367};
t2183 = ct{368};
t2184 = ct{369};
t2187 = ct{370};
t2189 = ct{371};
t2191 = ct{372};
t2193 = ct{373};
t2194 = ct{374};
t2201 = ct{375};
t2203 = ct{376};
t2205 = ct{377};
t2208 = ct{378};
t2210 = ct{379};
t2211 = ct{380};
t2212 = ct{381};
t2214 = ct{382};
t2216 = ct{383};
t2221 = ct{384};
t2223 = ct{385};
t2225 = ct{386};
t2229 = ct{387};
t223 = ct{388};
t2231 = ct{389};
t2232 = ct{390};
t2234 = ct{391};
t2235 = ct{392};
t2237 = ct{393};
t2239 = ct{394};
t2244 = ct{395};
t2246 = ct{396};
t225 = ct{397};
t2254 = ct{398};
t2258 = ct{399};
t2259 = ct{400};
t2261 = ct{401};
t2263 = ct{402};
t2264 = ct{403};
t2266 = ct{404};
t2267 = ct{405};
t2269 = ct{406};
t227 = ct{407};
t2271 = ct{408};
t2272 = ct{409};
t2273 = ct{410};
t228 = ct{411};
t2281 = ct{412};
t2285 = ct{413};
t2287 = ct{414};
t2288 = ct{415};
t2289 = ct{416};
t2290 = ct{417};
t2299 = ct{418};
t2309 = ct{419};
t231 = ct{420};
t2311 = ct{421};
t2313 = ct{422};
t2314 = ct{423};
t2315 = ct{424};
t2318 = ct{425};
t2320 = ct{426};
t2322 = ct{427};
t2323 = ct{428};
t2331 = ct{429};
t2332 = ct{430};
t2334 = ct{431};
t2335 = ct{432};
t2337 = ct{433};
t2339 = ct{434};
t2340 = ct{435};
t2341 = ct{436};
t2343 = ct{437};
t2344 = ct{438};
t2345 = ct{439};
t2347 = ct{440};
t2348 = ct{441};
t2351 = ct{442};
t2354 = ct{443};
t2355 = ct{444};
t236 = ct{445};
t2361 = ct{446};
t2362 = ct{447};
t2363 = ct{448};
t2364 = ct{449};
t2366 = ct{450};
t2367 = ct{451};
t2370 = ct{452};
t2376 = ct{453};
t2377 = ct{454};
t2378 = ct{455};
t2379 = ct{456};
t2380 = ct{457};
t2384 = ct{458};
t2390 = ct{459};
t2391 = ct{460};
t2393 = ct{461};
t2397 = ct{462};
t2401 = ct{463};
t2406 = ct{464};
t2409 = ct{465};
t2413 = ct{466};
t2415 = ct{467};
t2416 = ct{468};
t2418 = ct{469};
t2419 = ct{470};
t2421 = ct{471};
t2423 = ct{472};
t2425 = ct{473};
t2427 = ct{474};
t2430 = ct{475};
t2434 = ct{476};
t2435 = ct{477};
t2436 = ct{478};
t2439 = ct{479};
t2440 = ct{480};
t2441 = ct{481};
t2442 = ct{482};
t2443 = ct{483};
t2444 = ct{484};
t2445 = ct{485};
t2446 = ct{486};
t2447 = ct{487};
t2450 = ct{488};
t2451 = ct{489};
t2453 = ct{490};
t2454 = ct{491};
t2459 = ct{492};
t246 = ct{493};
t2461 = ct{494};
t2462 = ct{495};
t2467 = ct{496};
t2469 = ct{497};
t2472 = ct{498};
t2473 = ct{499};
t2475 = ct{500};
t2476 = ct{501};
t2478 = ct{502};
t2479 = ct{503};
t2489 = ct{504};
t2491 = ct{505};
t2505 = ct{506};
t2506 = ct{507};
t2507 = ct{508};
t2517 = ct{509};
t252 = ct{510};
t2523 = ct{511};
t2530 = ct{512};
t2531 = ct{513};
t2536 = ct{514};
t2537 = ct{515};
t2541 = ct{516};
t2542 = ct{517};
t2545 = ct{518};
t2546 = ct{519};
t2549 = ct{520};
t2550 = ct{521};
t2551 = ct{522};
t2553 = ct{523};
t2554 = ct{524};
t2555 = ct{525};
t2558 = ct{526};
t2559 = ct{527};
t2560 = ct{528};
t2565 = ct{529};
t2569 = ct{530};
t257 = ct{531};
t2576 = ct{532};
t2581 = ct{533};
t2583 = ct{534};
t2586 = ct{535};
t2588 = ct{536};
t2590 = ct{537};
t2592 = ct{538};
t2594 = ct{539};
t2596 = ct{540};
t2597 = ct{541};
t2603 = ct{542};
t2604 = ct{543};
t2605 = ct{544};
t2606 = ct{545};
t2616 = ct{546};
t2617 = ct{547};
t2618 = ct{548};
t2619 = ct{549};
t2620 = ct{550};
t2621 = ct{551};
t2625 = ct{552};
t2630 = ct{553};
t2631 = ct{554};
t2633 = ct{555};
t2650 = ct{556};
t2655 = ct{557};
t2661 = ct{558};
t2664 = ct{559};
t2667 = ct{560};
t2681 = ct{561};
t2683 = ct{562};
t2690 = ct{563};
t2691 = ct{564};
t2695 = ct{565};
t2697 = ct{566};
t2698 = ct{567};
t2702 = ct{568};
t2706 = ct{569};
t2708 = ct{570};
t2710 = ct{571};
t2711 = ct{572};
t2712 = ct{573};
t2718 = ct{574};
t2721 = ct{575};
t2722 = ct{576};
t2724 = ct{577};
t2725 = ct{578};
t2727 = ct{579};
t2728 = ct{580};
t273 = ct{581};
t2733 = ct{582};
t2736 = ct{583};
t2745 = ct{584};
t2747 = ct{585};
t2754 = ct{586};
t2755 = ct{587};
t2756 = ct{588};
t2762 = ct{589};
t2764 = ct{590};
t2766 = ct{591};
t2768 = ct{592};
t277 = ct{593};
t2770 = ct{594};
t2772 = ct{595};
t2775 = ct{596};
t2776 = ct{597};
t2777 = ct{598};
t2778 = ct{599};
t2779 = ct{600};
t2780 = ct{601};
t2781 = ct{602};
t2783 = ct{603};
t2784 = ct{604};
t2785 = ct{605};
t2786 = ct{606};
t2788 = ct{607};
t2789 = ct{608};
t2790 = ct{609};
t2792 = ct{610};
t300 = ct{611};
t308 = ct{612};
t31 = ct{613};
t311 = ct{614};
t312 = ct{615};
t313 = ct{616};
t314 = ct{617};
t315 = ct{618};
t32 = ct{619};
t328 = ct{620};
t33 = ct{621};
t333 = ct{622};
t342 = ct{623};
t346 = ct{624};
t36 = ct{625};
t395 = ct{626};
t396 = ct{627};
t397 = ct{628};
t451 = ct{629};
t452 = ct{630};
t455 = ct{631};
t470 = ct{632};
t485 = ct{633};
t5 = ct{634};
t500 = ct{635};
t51 = ct{636};
t515 = ct{637};
t53 = ct{638};
t533 = ct{639};
t544 = ct{640};
t55 = ct{641};
t565 = ct{642};
t57 = ct{643};
t580 = ct{644};
t6 = ct{645};
t614 = ct{646};
t639 = ct{647};
t648 = ct{648};
t654 = ct{649};
t655 = ct{650};
t66 = ct{651};
t671 = ct{652};
t673 = ct{653};
t675 = ct{654};
t679 = ct{655};
t68 = ct{656};
t7 = ct{657};
t703 = ct{658};
t710 = ct{659};
t711 = ct{660};
t717 = ct{661};
t725 = ct{662};
t726 = ct{663};
t727 = ct{664};
t748 = ct{665};
t75 = ct{666};
t765 = ct{667};
t769 = ct{668};
t770 = ct{669};
t773 = ct{670};
t788 = ct{671};
t795 = ct{672};
t8 = ct{673};
t822 = ct{674};
t826 = ct{675};
t836 = ct{676};
t854 = ct{677};
t856 = ct{678};
t865 = ct{679};
t87 = ct{680};
t873 = ct{681};
t888 = ct{682};
t889 = ct{683};
t890 = ct{684};
t896 = ct{685};
t9 = ct{686};
t902 = ct{687};
t909 = ct{688};
t910 = ct{689};
t914 = ct{690};
t929 = ct{691};
t930 = ct{692};
t933 = ct{693};
t938 = ct{694};
t942 = ct{695};
t944 = ct{696};
t969 = ct{697};
t977 = ct{698};
t979 = ct{699};
t98 = ct{700};
t980 = ct{701};
t2787 = t2134+t2174+t2176+t2225+t2281+t2285+t2415+t2423+t2453+t2517+t2583+t2661+t2664+t2667+t2681+t2754+t2756;
t2793 = t1972+t2008+t2011+t2013+t2054+t2055+t2131+t2141+t2164+t2187+t2210+t2214+t2239+t2309+t2323+t2363+t2366+t2397+t2409+t2419+t2427+t2441+t2443+t2536+t2546+t2549+t2553+t2586+t2592+t2698+t2708+t2710+t2727+t2762+t2766;
t2795 = t2004+t2005+t2056+t2066+t2070+t2073+t2094+t2107+t2109+t2128+t2135+t2194+t2229+t2232+t2258+t2266+t2313+t2318+t2332+t2339+t2351+t2370+t2390+t2393+t2430+t2439+t2442+t2467+t2472+t2489+t2530+t2531+t2569+t2625+t2631+t2650+t2690+t2691+t2745;
t2796 = t1671+t1687+t1784+t1785+t1867+t1991+t1992+t2095+t2098+t2101+t2114+t2118+t2139+t2142+t2201+t2208+t2212+t2221+t2223+t2237+t2259+t2264+t2334+t2337+t2343+t2348+t2355+t2364+t2384+t2391+t2434+t2440+t2445+t2469+t2473+t2491+t2537+t2541+t2576+t2630+t2633+t2655+t2695+t2697+t2747;
t2782 = t2231+t2290+t2299+t2545+t2560+t2603+t2683+t2755;
t2791 = t2047+t2090+t2093+t2129+t2166+t2170+t2244+t2246+t2261+t2289+t2314+t2322+t2416+t2459+t2505+t2506+t2507+t2523+t2581+t2588+t2706+t2721+t2724+t2725+t2768+t2775;
t2794 = t2017+t2024+t2029+t2041+t2077+t2080+t2148+t2152+t2156+t2193+t2205+t2216+t2271+t2331+t2341+t2354+t2361+t2401+t2418+t2421+t2425+t2444+t2446+t2542+t2551+t2554+t2558+t2590+t2597+t2702+t2711+t2712+t2736+t2764+t2770;
t2797 = t1789+t1969+t1970+t1996+t2021+t2025+t2059+t2068+t2079+t2089+t2111+t2112+t2161+t2203+t2211+t2234+t2235+t2263+t2311+t2315+t2320+t2340+t2344+t2347+t2362+t2367+t2435+t2436+t2447+t2450+t2451+t2454+t2550+t2555+t2559+t2565+t2594+t2596+t2718+t2722+t2728+t2733+t2772+t2776;
et213 = t31.*1.0e-4+t32.*1.0e-4;
et214 = t33.*5.582083966615414e-19+t36.*5.582083966615414e-19;
et215 = t31.*5.582083966615414e-19+t32.*5.582083966615414e-19+t33.*3.199999999999801e-4;
et216 = t36.*3.199999999999801e-4;
et217 = t119.*(et213+et214)-t1149.*(t342.*1.12e-3-t1168+t1213+t1232-t1337+t1365)+t2162.*(t312+t121.*(t51-t155))+t2267.*(t822+t228.*(t156-t236))+t2413.*(t1333+t888.*(t156-t236));
et218 = t902.*(t342.*3.844e-2-t1194+t1222+t1250-t1292+t1324);
et219 = (t1743+t1368.*(t485+t7.*(t53-t132))).*(t1901+t1906+t1974-t1975+t1368.*(t485+t7.*(t53-t132)).*7.950000000000001e-3+t1383.*(t485+t7.*(t53-t132)).*2.2e-4);
et220 = t314.*t2075+t313.*t2081+t1465.*t2254+t1966.*t2406+t654.*(-t909+t910+t929+t938+t1079+t1119);
et221 = t2069.*(t1893+t1904+t1980-t1981+t1368.*(t485+t7.*(t53-t132)).*2.900000000000001e-4+t1383.*(t485+t7.*(t53-t132)).*2.9e-4);
et222 = sin(q1+atan(2.19375)).^2.*5.8743807581e-5;
et223 = (-t98+t173+t580-t703-t930+t942-t9.*t10.*(2.1e+1./5.0e+1)+t7.*(t53-t132).*2.019e-2+t14.*(t53-t132).*4.9e-4).^2.*3.38795;
et224 = (t16+t18).*(t16.*2.9e-4+t18.*2.9e-4);
et225 = -t1627.*(-t1269+t1284+t1417+t1529+t228.*(t156-t236).*9.999999999999998e-6+t451.*(t156-t236).*1.2e-4);
et226 = (t1752+t1383.*(t485+t7.*(t53-t132))).*(t1896+t1903+t1976-t1977+t1368.*(t485+t7.*(t53-t132)).*2.2e-4+t1383.*(t485+t7.*(t53-t132)).*1.089e-2);
et227 = t120.*(et215+et216)+sin(q1-atan(4.558404558404559e-1)).^2.*5.8743807581e-5+t1327.^2.*4.50275+t1340.^2.*4.50275+t1771.^2.*2.4552+t1777.^2.*2.4552+t1949.^2.*2.61155;
et228 = t1960.^2.*2.61155+t1983.^2.*(3.41e+2./1.0e+2)+t1985.^2.*(3.41e+2./1.0e+2)+t2033.^2.*3.38795+t2126.^2.*3.5432e-1+t2136.^2.*3.5432e-1;
et229 = -t1826.*(t1662+t1665-t1772+t1773+t856.*(t156-t236).*2.81e-3+t888.*(t156-t236).*5.0e-5);
et230 = t1394.*4.000000000000028e-5+t1518+t1530+t1593+t1709+t565.*(t129+t13.*(t51-t155)).*5.0e-5;
et231 = t225.*(t136-t246).*2.81e-3+t452.*(t57-t165).*5.0e-5;
et232 = t856.*(t66-t210).*2.81e-3;
et233 = t17.*4.200000000000139e-4+t68.*4.200000000000139e-4;
et234 = t75.*4.200000000000139e-4;
et235 = t1537+t1575+t1704-t1710+t396.*(t167+t7.*(t55-t130)).*3.0e-5+t565.*(t129+t13.*(t51-t155)).*5.000000000000004e-4;
et236 = t225.*(t136-t246).*5.0e-5+t452.*(t57-t165).*5.000000000000004e-4;
et237 = t856.*(t66-t210).*5.0e-5;
et238 = sin(q2+atan(4.601355810186573e-2)).^2.*1.2537630455875e-1+t252.*t2184-t470.*t2191-t544.*t2183+t1505.*t2380+t1526.*t2378+t1757.*t2376+t1990.*t2479+t2035.*t2620;
et239 = (-t231+t397+t170.*(t53-t132)).*(t308.*1.11e-3+t977-t1033+t1095-t1136-t1155+t1159+t1300+t170.*(t53-t132).*4.988e-2);
et240 = (t1189+t225.*(t136-t246)+t856.*(t66-t210)).*(et230+et231+et232)-t2619.*(-t1614+t1626+t452.*(t515+t15.*(t57-t165)))-t2621.*(t1780-t1790+t889.*(t8.*(t57-t165)+t15.*(t136-t246)))+t223.*(et233+et234);
et241 = t933.*(t308.*1.144e-2-t1039-t1066+t1080-t1125+t1151+t1182+t1229+t170.*(t53-t132).*1.11e-3)+t979.^2.*4.50275;
et242 = t980.^2.*4.50275+t1366.^2.*2.4552+t1403.^2.*2.4552+t1404.^2.*2.4552+t1797.^2.*2.61155+t1808.^2.*2.61155+t1810.^2.*2.61155+t1919.^2.*(3.41e+2./1.0e+2)+t1953.^2.*(3.41e+2./1.0e+2)+t1954.^2.*(3.41e+2./1.0e+2)+t1993.^2.*3.38795+t2000.^2.*3.38795+t2001.^2.*3.38795+t2036.^2.*3.5432e-1;
et243 = t2065.^2.*3.5432e-1+t2067.^2.*3.5432e-1+(t1107+t565.*(t129+t13.*(t51-t155))+t452.*(t57-t165)).*(et235+et236+et237);
et244 = -t914.*(t308.*8.8e-4-t1020+t1034-t1094-t1124+t1131+t1140+t1255+t170.*(t53-t132).*1.12e-3);
et245 = t748.*2.81e-3+t1342-t1432+t1606+t1621-t1736+t648.*(t129+t13.*(t51-t155)).*5.0e-5;
et246 = t888.*(t153+t7.*(t143-t164)).*4.000000000000028e-5+t673.*(t156-t236).*5.0e-5;
et247 = t2478.*(t639+t648.*(t129+t13.*(t51-t155))+t673.*(t156-t236))+t346.*t2048+t455.*t2043+t500.*t2269+t1501.*t2377+t1504.*t2379+t1986.*t2476-t2032.*t2618+t2049.*t2616+t2121.*t2617+(t203-t679+t725.*2.324e-2+t865+t873+t1146+t14.*(t143-t164).*1.9738e-1).^2.*3.5432e-1-t2273.*(t180-t333+t5.*t121.*(t53-t132));
et248 = -t1769.*(t896-t1090+t1197+t1198+t1272-t1338-t1523+t300.*(t53-t132).*9.999999999999998e-6+t315.*(t156-t236).*1.2e-4)+t944.^2.*2.4552;
et249 = t1410.^2.*2.61155+t1568.^2.*2.4552+t1569.^2.*2.4552+t1699.^2.*2.61155+t1715.^2.*2.61155+t1782.^2.*(3.41e+2./1.0e+2)+t1883.^2.*(3.41e+2./1.0e+2)+t1885.^2.*(3.41e+2./1.0e+2)+t1965.^2.*3.38795+t1997.^2.*3.5432e-1+t1999.^2.*3.38795+t2002.^2.*3.38795+t2082.^2.*3.5432e-1+t1929.*(et245+et246);
et250 = -t2272.*(t191-t311+t122.*(t51-t155));
et251 = t2113.*(t1550-t1633-t1760+t1856+t1878-t1931-t1948+t1060.*(t485+t7.*(t53-t132)).*2.900000000000001e-4+t888.*(t257+t15.*(t273+t14.*(t51-t155))).*2.900000000000001e-4);
et252 = -1.0;
et253 = t1364-t1396+t1475-t1552+t671.*(t129+t13.*(t51-t155)).*5.000000000000004e-4+t655.*(t485+t7.*(t53-t132)).*3.0e-5;
et254 = t888.*(t273+t14.*(t51-t155)).*3.0e-5+t614.*(t156-t236).*5.000000000000004e-4;
et255 = t13.*t836.*(t53-t132).*5.0e-5;
et256 = t1560-t1637-t1754+t1857+t1879-t1927-t1943+t1060.*(t485+t7.*(t53-t132)).*7.950000000000001e-3;
et257 = t888.*(t257+t15.*(t273+t14.*(t51-t155))).*7.950000000000001e-3;
et258 = t710.*4.000000000000028e-5-t1375+t1486+t1535+t1542+t671.*(t129+t13.*(t51-t155)).*3.0e-5;
et259 = t655.*(t485+t7.*(t53-t132)).*2.32e-3+t888.*(t273+t14.*(t51-t155)).*2.32e-3;
et260 = t614.*(t156-t236).*3.0e-5;
et261 = et251.*et252+(-t87-t172+t277.*4.9e-4+t711+t727+t770+t13.*(t53-t132).*2.75e-2).^2.*3.38795+t773.*t2133-t1097.*t2122-t1603.*t2345-t1658.*t2335+t1884.*t2475;
et262 = t2051.*(t1546-t1632-t1749+t1855+t1877-t1926-t1944+t1060.*(t485+t7.*(t53-t132)).*2.2e-4+t888.*(t257+t15.*(t273+t14.*(t51-t155))).*2.2e-4);
et263 = (-t726+t671.*(t129+t13.*(t51-t155))+t614.*(t156-t236)).*(et253+et254+et255)+(t1120+t1060.*(t485+t7.*(t53-t132))+t888.*(t257+t15.*(t273+t14.*(t51-t155)))).*(et256+et257);
et264 = t854.*(t969+t1116+t1117+t1183-t1204-t1414-t1419+t451.*(t51-t155).*1.0e-5+t6.*t228.*(t129+t13.*(t51-t155)).*9.999999999999998e-6)+t1601.^2.*2.61155;
et265 = t1625.^2.*(3.41e+2./1.0e+2)+t1707.^2.*2.61155+t1731.^2.*2.61155+t1776.^2.*(3.41e+2./1.0e+2)+t1783.^2.*(3.41e+2./1.0e+2)+t1935.^2.*3.38795+t2007.^2.*3.5432e-1+t2057.^2.*3.5432e-1+t2072.^2.*3.5432e-1+(t890+t655.*(t485+t7.*(t53-t132))+t888.*(t273+t14.*(t51-t155))).*(et258+et259+et260);
et266 = (t112+t205+t717+t765-t769+t7.*(t51-t155).*2.019e-2+t14.*(t51-t155).*4.9e-4).^2.*3.38795;
et267 = -t1584+t1604+t1823+t1839-t1942-t1957+t675.*(t8.*(t57-t165)+t15.*(t136-t246)).*2.9e-4+t14.*t1383.*(t129+t13.*(t51-t155)).*1.089e-2;
et268 = t14.*t1359.*(t156-t236).*1.089e-2;
et269 = -t1595+t1607+t1828+t1851-t1940-t1955+t675.*(t8.*(t57-t165)+t15.*(t136-t246)).*2.900000000000001e-4+t14.*t1383.*(t129+t13.*(t51-t155)).*2.2e-4;
et270 = t14.*t1359.*(t156-t236).*2.2e-4;
et271 = -t1589+t1605+t1819+t1831-t1946-t1963+t675.*(t8.*(t57-t165)+t15.*(t136-t246)).*2.94e-3+t14.*t1383.*(t129+t13.*(t51-t155)).*2.9e-4;
et272 = t14.*t1359.*(t156-t236).*2.9e-4;
et273 = (t1203+t14.*t1383.*(t129+t13.*(t51-t155))+t14.*t1359.*(t156-t236)).*(et267+et268);
et274 = t1398.*(t1132+t1293+t1312+t1425-t1629-t1645-t1648+t227.*(t136-t246).*5.0e-5+t7.*t888.*(t129+t13.*(t51-t155)).*3.0e-5);
et275 = -(et269+et270).*(t1179-t1618+t1105.*(t485+t7.*(t53-t132)))+t1341.*t2189-t1967.*t2462-t1973.*t2461-t2120.*(et271+et272)+t1697.^2.*(3.41e+2./1.0e+2)+t1802.^2.*3.38795+t1803.^2.*(3.41e+2./1.0e+2)+t1805.^2.*(3.41e+2./1.0e+2)+t1930.^2.*3.38795+t1945.^2.*3.38795+t1987.^2.*3.5432e-1+t2019.^2.*3.5432e-1+t2027.^2.*3.5432e-1-t2175.*(t328-t795+t395.*(t53-t132));
et276 = -t1766+t396.*(t515+t15.*(t57-t165))+t1359.*(t485+t7.*(t53-t132));
et277 = t1499+t1711+t1726-t1924+t396.*(t515+t15.*(t57-t165)).*7.950000000000001e-3+t1359.*(t485+t7.*(t53-t132)).*7.950000000000001e-3;
et278 = (t533.*2.324e-2+t788+t8.*(t57-t165).*3.466000000000001e-2+t15.*(t136-t246).*3.466000000000001e-2).^2.*3.5432e-1+et276.*et277+t2009.^2.*3.5432e-1+t2016.^2.*3.5432e-1;
et279 = t1984.*(t1507+t1719+t1741-t1923+t396.*(t515+t15.*(t57-t165)).*2.900000000000001e-4+t1359.*(t485+t7.*(t53-t132)).*2.900000000000001e-4);
mt1 = [et217+et218+et219+et220+et221+et222+et223+et224+et225+et226+et227+et228+et229,t2796,t2795,t2792,t2788,t2783,t2777,t2796,et238+et239+et240+et241+et242+et243+et244,t2797,t2794,t2791,t2787,t2782,t2795,t2797,et247+et248+et249+et250,t2793,t2790,t2786,t2781,t2792,t2794,t2793,et261+et262+et263+et264+et265+et266,t2789,t2785,t2780,t2788,t2791,t2790,t2789,et273+et274+et275,t2784,t2779,t2783,t2787,t2786,t2785,t2784];
mt2 = [t1738.*t2288+t1768.*t2606+t2084.*t2604+t2088.*t2605+t2287.*(-t826+t856.*(t129+t13.*(t51-t155))+t836.*(t156-t236))+t1804.^2.*3.38795+t1952.^2.*3.38795+t1961.^2.*3.5432e-1+t1964.^2.*3.38795+t2003.^2.*3.5432e-1+t2006.^2.*3.5432e-1,t2778,t2777,t2782,t2781,t2780,t2779,t2778,et278+et279];
M = reshape([mt1,mt2],7,7);
end
